simulink model "Supplementary_With_Disturbance"  (R2021a)
(part 42 of 51)

                                                                                                                                                                                                                                                                                                                                                                                                                                                                                                                                                                                                                                                                                                                                                                                                                                                                                                                                                                                                                                                                                                                                                                                                                                                                                                                                                                                                                                                                                                                                                                                                                                                                                                                                                                                                                                                                                                                                                                                                                                                                                                                                                                                                                                                                                                                                                                                                                                                                                                                                                                                                                                                                                                                                                                                                                                                                                                                                                                                                                                                                                                                                                                                                                                                                                                                                                                                                                                                                                                                                                                                                                                                                                                                                                                                                                                                                                                                                                                                                                                                                                                                                                                                                                                                                                                                                                                                                                                                                                                                                                                                                                                                                                                                                                                                                                                                                                                                                                                                                                                                                                                                                                                                                                                                                                                                                                                                                                                                                                                                                                                                                                                                                                                                                                                                                                                                                                                                                                                                                                                                                                                                                                                                                                                                                                                                                                                                                                                                                                                                                                                                                                                                                                                                                                                                                                                                                                                                                                                                                                                                                                                                                                                                                                                                                                                                                                                                                                                                                                                                                                                                                                                                                                                                                                                                                                                                                                                                                                                                                                                                                                                                                                                                                                                                                                                                                                                                                                                                                                                                                                                                                                                                                                                                                                                                                                                                                                                                                                                                                                                                                                                                                                                                                                                                                                                                                                                                                                                                                                                                                                                                                                                                                                                                                                                                                                                                                                                                                                                                                                                                                                                                                                                                                                                                                                                                                                                                                                                                                                                                                                                                                                                                                                                                                                                                                                                                                                                                                                                                                             0.5*I_yz_4*cos(theta3 - theta2 + theta4) + (I_xz_4*sin(theta3 - theta2 + theta4))/2 - 0.5*I_xz_5*cos(theta2 + theta3 + theta4 + theta5) + 0.5*I_yz_5*sin(theta2 + theta3 + theta4 + theta5) + I_zz_4*sin(theta2) + I_zz_5*sin(theta2) - 0.5*I_xz_5*cos(theta3 - theta2 + theta4 + theta5) + 0.5*I_yz_5*sin(theta3 - theta2 + theta4 + theta5) + 0.5*I_yz_4*cos(theta2 + theta3 + theta4) + (I_xz_4*sin(theta2 + theta3 + theta4))/2 + 0.25*a4^2*m4*sin(theta2) + a4^2*m5*sin(theta2) + 0.25*a5^2*m5*sin(theta2) + lc4_1^2*m4*sin(theta2) + lc4_2^2*m4*sin(theta2) + lc5_1^2*m5*sin(theta2) + lc5_2^2*m5*sin(theta2) - 0.25*a2*a4*m4*cos(theta3 - theta2 + theta4) - 0.5*a2*a4*m5*cos(theta3 - theta2 + theta4) + 0.25*a3*a5*m5*cos(theta4 - theta2 + theta5) - 0.5*a2*lc4_1*m4*cos(theta3 - theta2 + theta4) + (a3*lc5_1*m5*cos(theta4 - theta2 + theta5))/2 - 0.5*lc4_2*lc4_3*m4*cos(theta3 - theta2 + theta4) + 0.5*a2*lc4_2*m4*sin(theta3 - theta2 + theta4) - 0.25*a4*lc4_3*m4*sin(theta3 - theta2 + theta4) - 0.5*a3*lc5_2*m5*sin(theta4 - theta2 + theta5) - 0.5*a4*lc5_3*m5*sin(theta3 - theta2 + theta4) + 0.5*a2*lc5_2*m5*cos(theta2 + theta3 + theta4 + theta5) + 0.25*a5*lc5_3*m5*cos(theta2 + theta3 + theta4 + theta5) + 0.25*a2*a5*m5*sin(theta2 + theta3 + theta4 + theta5) - 0.5*lc4_1*lc4_3*m4*sin(theta3 - theta2 + theta4) + 0.5*lc5_1*lc5_3*m5*cos(theta2 + theta3 + theta4 + theta5) - (a4*a5*m5*cos(theta2 + theta5))/2 + 0.5*a2*lc5_1*m5*sin(theta2 + theta3 + theta4 + theta5) - 1.0*a1*lc4_2*m4*cos(theta3 + theta4) + 0.5*a3*lc4_2*m4*cos(theta2 + theta4) - 1.0*a4*lc5_1*m5*cos(theta2 + theta5) - 0.5*lc5_2*lc5_3*m5*sin(theta2 + theta3 + theta4 + theta5) - 0.5*a1*a4*m4*sin(theta3 + theta4) - 1.0*a1*a4*m5*sin(theta3 + theta4) + 0.25*a3*a4*m4*sin(theta2 + theta4) + (a3*a4*m5*sin(theta2 + theta4))/2 - 1.0*a1*lc4_1*m4*sin(theta3 + theta4) + (a3*lc4_1*m4*sin(theta2 + theta4))/2 + 1.0*a4*lc5_2*m5*sin(theta2 + theta5) + a4*lc4_1*m4*sin(theta2) + a5*lc5_1*m5*sin(theta2) - 0.5*a2*lc5_2*m5*cos(theta3 - theta2 + theta4 + theta5) + 0.25*a5*lc5_3*m5*cos(theta3 - theta2 + theta4 + theta5) - 0.25*a2*a5*m5*sin(theta3 - theta2 + theta4 + theta5) + 0.5*lc5_1*lc5_3*m5*cos(theta3 - theta2 + theta4 + theta5) + (a4*a5*m5*cos(theta2 - theta5))/2 - 0.5*a2*lc5_1*m5*sin(theta3 - theta2 + theta4 + theta5) - 0.5*a3*lc4_2*m4*cos(theta2 - theta4) + 1.0*a4*lc5_1*m5*cos(theta2 - theta5) - 0.5*lc5_2*lc5_3*m5*sin(theta3 - theta2 + theta4 + theta5) + 0.25*a3*a4*m4*sin(theta2 - theta4) + (a3*a4*m5*sin(theta2 - theta4))/2 + 0.25*a2*a4*m4*cos(theta2 + theta3 + theta4) + 0.5*a2*a4*m5*cos(theta2 + theta3 + theta4) + 0.5*a1*a5*m5*cos(theta3 + theta4 + theta5) - 0.25*a3*a5*m5*cos(theta2 + theta4 + theta5) + (a3*lc4_1*m4*sin(theta2 - theta4))/2 + 1.0*a4*lc5_2*m5*sin(theta2 - theta5) + 0.5*a2*lc4_1*m4*cos(theta2 + theta3 + theta4) + 1.0*a1*lc5_1*m5*cos(theta3 + theta4 + theta5) - (a3*lc5_1*m5*cos(theta2 + theta4 + theta5))/2 - 0.5*lc4_2*lc4_3*m4*cos(theta2 + theta3 + theta4) - 0.5*a2*lc4_2*m4*sin(theta2 + theta3 + theta4) - 0.25*a4*lc4_3*m4*sin(theta2 + theta3 + theta4) - 1.0*a1*lc5_2*m5*sin(theta3 + theta4 + theta5) + 0.5*a3*lc5_2*m5*sin(theta2 + theta4 + theta5) - 0.5*a4*lc5_3*m5*sin(theta2 + theta3 + theta4) - 0.5*lc4_1*lc4_3*m4*sin(theta2 + theta3 + theta4),                                                                                                                                                                                                                                                                                                                                                                                                                                                                                                                                                                                                                                                                                                                                                                                                                                                                                                                                                                                                                                                                                                                                                                                                                                                                                                                                                                                                                                                                                                                                                                                                                                                                                                                                                                                                                                                                                                                                                                                                                                                                                                                                                                                                                                                                                                                                                                                                                                                                                                                                                                                                                                                                                                                                                                                                                                                                                                                                                                                                                                                                                                                                                                                                                                                                                                                                                                                                                                                                                                                                                                                                                                                                                                                                                                                                                                                                                                                                                                                                                                                                                                                                                                                                                                                                                                                                                                                                                                                                                                                                                                                                                                                                                                                                                                                                                                                                                                                                                                                                                                                                                                                                                                                                                                                                                                                                                                                                                                                                                                                                                                                                                                                                                                                                                                                                                                                                                                                                                                                                                                                                                                                                                                                                                                                                                                                                                                                                                                                                                                                                                                                                                                                                                                                                                                                                                 I_yz_4*sin(theta3 + theta4) - 1.0*I_xz_4*cos(theta3 + theta4) - 1.0*I_yz_5*cos(theta3 + theta4 + theta5) - 1.0*I_xz_5*sin(theta3 + theta4 + theta5) + 0.5*a4*lc4_3*m4*cos(theta3 + theta4) + a4*lc5_3*m5*cos(theta3 + theta4) + lc4_1*lc4_3*m4*cos(theta3 + theta4) - 1.0*lc4_2*lc4_3*m4*sin(theta3 + theta4) + lc5_2*lc5_3*m5*cos(theta3 + theta4 + theta5) + 0.5*a5*lc5_3*m5*sin(theta3 + theta4 + theta5) + lc5_1*lc5_3*m5*sin(theta3 + theta4 + theta5),                                                                                                                                                                                                                                                                                                                                                                                                                                                                                                                                                                                                                                                                                                                                                                                                                                                                                                                                                                                                                                                                                                                                                                                                                                                                                                                                                                                                                                                                                                                                                                                                                                                                                                                                                                                                                                                                                                                                                                                                                                                                                                                                                                                                                                                                                                                                                                                                                                                                                                                                                                                                                                                                                                                                                                                                                                                                                                                                                                                                                                                                                                                                                                                                                                                                                                                                                                                                                                                                                                                                                                                                                                                                                                                                                                                                                                                                                                                                                                                                                                                                                                                  I_zz_4 + I_zz_5 + 0.25*a4^2*m4 + a4^2*m5 + 0.25*a5^2*m5 + lc4_1^2*m4 + lc4_2^2*m4 + lc5_1^2*m5 + lc5_2^2*m5 + a4*lc4_1*m4 + a5*lc5_1*m5 + a3*lc5_2*m5*cos(theta4 + theta5) + 0.5*a3*a5*m5*sin(theta4 + theta5) + a3*lc5_1*m5*sin(theta4 + theta5) + 0.5*a3*a4*m4*cos(theta4) + a3*a4*m5*cos(theta4) + a3*lc4_1*m4*cos(theta4) + 2.0*a4*lc5_2*m5*cos(theta5) + a4*a5*m5*sin(theta5) - 1.0*a3*lc4_2*m4*sin(theta4) + 2.0*a4*lc5_1*m5*sin(theta5),                                                                                                                                                                                                                                                                                                                                                                                                                                                                                                                                                                                                                                                                                                                                                                                                                                                                                                                                                                                                                                                                                                                                                                                                                                                                                                                                                                                                                                                                                                                                                                                                                                                                                                                                                                                                                                                                                                                                                                                                                                                                                                                                                                                                                                                                                                                                                                                                                                                                                                                                                                                                                                                                                                                                                                                                                                                                                                                                                                                                                                                                                                                         I_zz_4 + I_zz_5 + 0.25*a4^2*m4 + a4^2*m5 + 0.25*a5^2*m5 + lc4_1^2*m4 + lc4_2^2*m4 + lc5_1^2*m5 + lc5_2^2*m5 + a4*lc4_1*m4 + a5*lc5_1*m5 + 2.0*a4*lc5_2*m5*cos(theta5) + a4*a5*m5*sin(theta5) + 2.0*a4*lc5_1*m5*sin(theta5),                                                                                                                                                                                                                                                                                                                                                                                                                                                                                                                                                                                                                                                                                                                                                                                                                                                                                                                                                                                                                                                                                                                                                                                                                                                                                                                                                                                                                                                                                                                    0.25*m5*a5^2 + m5*a5*lc5_1 + 0.5*a4*m5*sin(theta5)*a5 + m5*lc5_1^2 + a4*m5*sin(theta5)*lc5_1 + m5*lc5_2^2 + a4*m5*cos(theta5)*lc5_2 + I_zz_5
                                                                                                                                                                                                                                                                                                                                                                                                                                                                                                                                                                                                                                                                                                                                                                                                                                                                                                                                                                                                                                                                                                                                                                                                                                                                                                                                                                                                                                                                                                                                                                                                                                                                                                                                                                                                                                                                                                                                                                                                                                                                                                                                                                                                                                                                                                                                                                                                                                                                                                                                                                                                                                                                                                                                                                                                                                                                                                                                                                                                                                                                                                                                                                                                                                                                                                                                                                                                                                                                                                                                                                                                                                                                                                                                                                                                                                                                                                                                                                                                                                                                                                                                                                                                                                                                                                                                                                                                                                                                                                                                                                                                                                                                                                                                                                                                                                                                                                                                                                                                                                                                                                                                                                                                                                                                                                                                                                                                                                                                                                                                                                                                                                                                                                                                                                                                                                                                                                                                                                                                                                                                                                                                                                                                                                                                                                                                                                                                                                                                                                                                                                                                                                                                                                                                                                                                                                                                                                                                                                                                                                                                                                                                                                                                                                                                                                                                                                                                                                                                                                                                                                                                                                                                                                                                                                                                                                                                                                                                                                                                                                                                                                                                                                                                                                                                                                                                                                                                                                                                                                                                                                                                                                                                                                                                                                                                                                                                                                                                                                                                                                                                                                                                                                                                                                                                                                                                                                                                                                                                                                                                                                                                                                                                                                                                                                                                                                                                                                                                                                                                                                                                                                                                                                                                                                                                                                                                                                                                                                                                                                                                                                                                                                                                                                                                                                                                                                                                                                                                                                                                                                                                                                                                                                                                                                                                                                                                                                                                                                                                                                                                                                                                                                                                                                                                                                                                                                                                                                                                                                                                                                                                                                                                                                                                                                                                                                                                                                                                                                                                                                                                                                                                                                                                                                0.5*I_yz_5*sin(theta2 + theta3 + theta4 + theta5) - 0.5*I_xz_5*cos(theta2 + theta3 + theta4 + theta5) + I_zz_5*sin(theta2) - 0.5*I_xz_5*cos(theta3 - theta2 + theta4 + theta5) + 0.5*I_yz_5*sin(theta3 - theta2 + theta4 + theta5) + 0.25*a5^2*m5*sin(theta2) + lc5_1^2*m5*sin(theta2) + lc5_2^2*m5*sin(theta2) + 0.25*a3*a5*m5*cos(theta4 - theta2 + theta5) + (a3*lc5_1*m5*cos(theta4 - theta2 + theta5))/2 - 0.5*a3*lc5_2*m5*sin(theta4 - theta2 + theta5) + 0.5*a2*lc5_2*m5*cos(theta2 + theta3 + theta4 + theta5) + 0.25*a5*lc5_3*m5*cos(theta2 + theta3 + theta4 + theta5) + 0.25*a2*a5*m5*sin(theta2 + theta3 + theta4 + theta5) + 0.5*lc5_1*lc5_3*m5*cos(theta2 + theta3 + theta4 + theta5) + 0.5*a2*lc5_1*m5*sin(theta2 + theta3 + theta4 + theta5) - 0.5*lc5_2*lc5_3*m5*sin(theta2 + theta3 + theta4 + theta5) + (a4*lc5_2*m5*sin(theta2 + theta5))/2 + a5*lc5_1*m5*sin(theta2) - 0.5*a2*lc5_2*m5*cos(theta3 - theta2 + theta4 + theta5) + 0.25*a5*lc5_3*m5*cos(theta3 - theta2 + theta4 + theta5) - 0.25*a2*a5*m5*sin(theta3 - theta2 + theta4 + theta5) + 0.5*lc5_1*lc5_3*m5*cos(theta3 - theta2 + theta4 + theta5) - 0.5*a2*lc5_1*m5*sin(theta3 - theta2 + theta4 + theta5) - 0.5*lc5_2*lc5_3*m5*sin(theta3 - theta2 + theta4 + theta5) + 0.5*a1*a5*m5*cos(theta3 + theta4 + theta5) - 0.25*a3*a5*m5*cos(theta2 + theta4 + theta5) + (a4*lc5_2*m5*sin(theta2 - theta5))/2 + a1*lc5_1*m5*cos(theta3 + theta4 + theta5) - (a3*lc5_1*m5*cos(theta2 + theta4 + theta5))/2 - 1.0*a1*lc5_2*m5*sin(theta3 + theta4 + theta5) + 0.5*a3*lc5_2*m5*sin(theta2 + theta4 + theta5) + 0.5*a4*a5*m5*sin(theta2)*sin(theta5) + a4*lc5_1*m5*sin(theta2)*sin(theta5),                                                                                                                                                                                                                                                                                                                                                                                                                                                                                                                                                                                                                                                                                                                                                                                                                                                                                                                                                                                                                                                                                                                                                                                                                                                                                                                                                                                                                                                                                                                                                                                                                                                                                                                                                                                                                                                                                                                                                                                                                                                                                                                                                                                                                                                                                                                                                                                                                                                                                                                                                                                                                                                                                                                                                                                                                                                                                                                                                                                                                                                                                                                                                                                                                                                                                                                                                                                                                                                                                                                                                                                                                                                                                                                                                                                                                                                                                                                                                                                                                                                                                                                                                                                                                                                                                                                                                                                                                                                                                                                                                                                                                                                                                                                                                                                                                                                                                                                                                                                                                                                                                                                                                                                                                                                                                                                                                                                                                                                                                                                                                                                                                                                                                                                                                                                                                                                                                                                                                                                                                                                                                                                                                                                                                                                                                                                                                                                                                                                                                                                                                                                                                                                                                                                                                                                                                                                                                                                                                                                                                                           lc5_2*lc5_3*m5*cos(theta3 + theta4 + theta5) - 1.0*I_xz_5*sin(theta3 + theta4 + theta5) - 1.0*I_yz_5*cos(theta3 + theta4 + theta5) + 0.5*a5*lc5_3*m5*sin(theta3 + theta4 + theta5) + lc5_1*lc5_3*m5*sin(theta3 + theta4 + theta5),                                                                                                                                                                                                                                                                                                                                                                                                                                                                                                                                                                                                                                                                                                                                                                                                                                                                                                                                                                                                                                                                                                                                                                                                                                                                                                                                                                                                                                                                                                                                                                                                                                                                                                                                                                                                                                                                                                                                                                                                                                                                                                                                                                                                                                                                                                                                                                                                                                                                                                                                                                                                                                                                                                                                                                                                                                                                                                                                                                                                                                                                                                                                                                                                                                                                                                                                                                                                                                                                                                                                                                                                                                                                                                                                                                                                                                                                                                                                                                                                                                                                                                                                                                                                                                                                                                          I_zz_5 + 0.25*a5^2*m5 + lc5_1^2*m5 + lc5_2^2*m5 + a5*lc5_1*m5 + a3*lc5_2*m5*cos(theta4 + theta5) + 0.5*a3*a5*m5*sin(theta4 + theta5) + a3*lc5_1*m5*sin(theta4 + theta5) + a4*lc5_2*m5*cos(theta5) + 0.5*a4*a5*m5*sin(theta5) + a4*lc5_1*m5*sin(theta5),                                                                                                                                                                                                                                                                                                                                                                                                                                                                                                                                                                                                                                                                                                                                                                                                                                                                                                                                                                                                                                                                                                                                                                                                                                                                                                                                                                                                                                                                                                                                                                                                                                                                                                                                                                                                                                                                                                                                                                                                                                                                                                                                                                                                                                                                                                                                                                                                                                                                                                                                                                                                                                                                                                                                                                                                                                                                                                                                                                                                                                                                                                                                                                                                       0.25*m5*a5^2 + m5*a5*lc5_1 + 0.5*a4*m5*sin(theta5)*a5 + m5*lc5_1^2 + a4*m5*sin(theta5)*lc5_1 + m5*lc5_2^2 + a4*m5*cos(theta5)*lc5_2 + I_zz_5,                                                                                                                                                                                                                                                                                                                                                                                                                                                                                                                                                                                                                                                                                                                                                                                                                                                                                                                                                                                                                                                                                                                                                                                                                                                                                                                                                                                                                                                                                                                                                                                                   0.25*m5*a5^2 + m5*a5*lc5_1 + m5*lc5_1^2 + m5*lc5_2^2 + I_zz_5]
 
%%%%%%%%%%%%%%%%%%%%%%%%%%%%%
% Coriolis and Centripetal Matrix
C11a = 0.5*I_yz_3*theta_dot_2*cos(2.0*theta2 - 1.0*theta3) - 0.25*I_yz_3*theta_dot_3*cos(2.0*theta2 - 1.0*theta3) - 0.5*I_xz_3*theta_dot_2*sin(2.0*theta2 - 1.0*theta3) + 0.25*I_xz_3*theta_dot_3*sin(2.0*theta2 - 1.0*theta3) - 0.25*I_xy_5*theta_dot_2*cos(2*theta2 + 2*theta3 + 2*theta4 + 2*theta5) - 0.25*I_xy_5*theta_dot_3*cos(2*theta2 + 2*theta3 + 2*theta4 + 2*theta5) - 0.25*I_xy_5*theta_dot_4*cos(2*theta2 + 2*theta3 + 2*theta4 + 2*theta5) - 0.25*I_xy_5*theta_dot_5*cos(2*theta2 + 2*theta3 + 2*theta4 + 2*theta5) - 0.125*I_xx_5*theta_dot_2*sin(2*theta2 + 2*theta3 + 2*theta4 + 2*theta5) - 0.125*I_xx_5*theta_dot_3*sin(2*theta2 + 2*theta3 + 2*theta4 + 2*theta5) - 0.125*I_xx_5*theta_dot_4*sin(2*theta2 + 2*theta3 + 2*theta4 + 2*theta5) - 0.125*I_xx_5*theta_dot_5*sin(2*theta2 + 2*theta3 + 2*theta4 + 2*theta5) + 0.125*I_yy_5*theta_dot_2*sin(2*theta2 + 2*theta3 + 2*theta4 + 2*theta5) + 0.125*I_yy_5*theta_dot_3*sin(2*theta2 + 2*theta3 + 2*theta4 + 2*theta5) + 0.125*I_yy_5*theta_dot_4*sin(2*theta2 + 2*theta3 + 2*theta4 + 2*theta5) + 0.125*I_yy_5*theta_dot_5*sin(2*theta2 + 2*theta3 + 2*theta4 + 2*theta5) - 0.5*I_xz_5*theta_dot_2*cos(theta3 - 2.0*theta2 + theta4 + theta5) - 0.5*I_xz_5*theta_dot_2*cos(2.0*theta2 + theta3 + theta4 + theta5) + 0.25*I_xz_5*theta_dot_3*cos(theta3 - 2.0*theta2 + theta4 + theta5) - 0.25*I_xz_5*theta_dot_3*cos(2.0*theta2 + theta3 + theta4 + theta5) + 0.25*I_xz_5*theta_dot_4*cos(theta3 - 2.0*theta2 + theta4 + theta5) - 0.25*I_xz_5*theta_dot_4*cos(2.0*theta2 + theta3 + theta4 + theta5) + 0.25*I_xz_5*theta_dot_5*cos(theta3 - 2.0*theta2 + theta4 + theta5) - 0.25*I_xz_5*theta_dot_5*cos(2.0*theta2 + theta3 + theta4 + theta5) + 0.25*I_xy_4*theta_dot_2*cos(2*theta2 + 2*theta3 + 2*theta4) + 0.25*I_xy_4*theta_dot_3*cos(2*theta2 + 2*theta3 + 2*theta4) + 0.25*I_xy_4*theta_dot_4*cos(2*theta2 + 2*theta3 + 2*theta4) - 0.5*I_xy_5*theta_dot_3*cos(2*theta3 + 2*theta4 + 2*theta5) - 0.5*I_xy_5*theta_dot_4*cos(2*theta3 + 2*theta4 + 2*theta5) - 0.5*I_xy_5*theta_dot_5*cos(2*theta3 + 2*theta4 + 2*theta5) + 0.5*I_yz_5*theta_dot_2*sin(theta3 - 2.0*theta2 + theta4 + theta5) + 0.5*I_yz_5*theta_dot_2*sin(2.0*theta2 + theta3 + theta4 + theta5) - 0.25*I_yz_5*theta_dot_3*sin(theta3 - 2.0*theta2 + theta4 + theta5) + 0.25*I_yz_5*theta_dot_3*sin(2.0*theta2 + theta3 + theta4 + theta5) - 0.25*I_yz_5*theta_dot_4*sin(theta3 - 2.0*theta2 + theta4 + theta5) + 0.25*I_yz_5*theta_dot_4*sin(2.0*theta2 + theta3 + theta4 + theta5) - 0.25*I_yz_5*theta_dot_5*sin(theta3 - 2.0*theta2 + theta4 + theta5) + 0.25*I_yz_5*theta_dot_5*sin(2.0*theta2 + theta3 + theta4 + theta5) + 0.5*I_yz_3*theta_dot_2*cos(2.0*theta2 + theta3) + 0.25*I_yz_3*theta_dot_3*cos(2.0*theta2 + theta3) + 0.125*I_xx_4*theta_dot_2*sin(2*theta2 + 2*theta3 + 2*theta4) + 0.125*I_xx_4*theta_dot_3*sin(2*theta2 + 2*theta3 + 2*theta4) + 0.125*I_xx_4*theta_dot_4*sin(2*theta2 + 2*theta3 + 2*theta4) - 0.25*I_xx_5*theta_dot_3*sin(2*theta3 + 2*theta4 + 2*theta5) - 0.25*I_xx_5*theta_dot_4*sin(2*theta3 + 2*theta4 + 2*theta5) - 0.25*I_xx_5*theta_dot_5*sin(2*theta3 + 2*theta4 + 2*theta5) - 0.125*I_yy_4*theta_dot_2*sin(2*theta2 + 2*theta3 + 2*theta4) - 0.125*I_yy_4*theta_dot_3*sin(2*theta2 + 2*theta3 + 2*theta4) - 0.125*I_yy_4*theta_dot_4*sin(2*theta2 + 2*theta3 + 2*theta4) + 0.25*I_yy_5*theta_dot_3*sin(2*theta3 + 2*theta4 + 2*theta5) + 0.25*I_yy_5*theta_dot_4*sin(2*theta3 + 2*theta4 + 2*theta5) + 0.25*I_yy_5*theta_dot_5*sin(2*theta3 + 2*theta4 + 2*theta5) + 0.5*I_xz_3*theta_dot_2*sin(2.0*theta2 + theta3) + 0.25*I_xz_3*theta_dot_3*sin(2.0*theta2 + theta3) + 0.25*I_xy_3*theta_dot_2*cos(2*theta2 + 2*theta3) + 0.25*I_xy_3*theta_dot_3*cos(2*theta2 + 2*theta3) + 0.5*I_xy_4*theta_dot_3*cos(2*theta3 + 2*theta4) + 0.5*I_xy_4*theta_dot_4*cos(2*theta3 + 2*theta4) - 1.0*I_xz_2*theta_dot_2*cos(2.0*theta2) + 0.5*I_xy_3*theta_dot_3*cos(2.0*theta3) + 0.125*I_xx_3*theta_dot_2*sin(2*theta2 + 2*theta3) + 0.125*I_xx_3*theta_dot_3*sin(2*theta2 + 2*theta3) + 0.25*I_xx_4*theta_dot_3*sin(2*theta3 + 2*theta4) + 0.25*I_xx_4*theta_dot_4*sin(2*theta3 + 2*theta4) - 0.125*I_yy_3*theta_dot_2*sin(2*theta2 + 2*theta3) - 0.125*I_yy_3*theta_dot_3*sin(2*theta2 + 2*theta3) - 0.25*I_yy_4*theta_dot_3*sin(2*theta3 + 2*theta4) - 0.25*I_yy_4*theta_dot_4*sin(2*theta3 + 2*theta4) - 0.5*I_xx_2*theta_dot_2*sin(2.0*theta2) - 0.25*I_xx_3*theta_dot_2*sin(2.0*theta2) - 0.25*I_xx_4*theta_dot_2*sin(2.0*theta2) + 0.25*I_xx_3*theta_dot_3*sin(2.0*theta3) - 0.25*I_xx_5*theta_dot_2*sin(2.0*theta2) - 0.25*I_yy_3*theta_dot_2*sin(2.0*theta2) - 0.25*I_yy_4*theta_dot_2*sin(2.0*theta2) - 0.25*I_yy_3*theta_dot_3*sin(2.0*theta3) - 0.25*I_yy_5*theta_dot_2*sin(2.0*theta2) + 0.5*I_zz_2*theta_dot_2*sin(2.0*theta2) + 0.5*I_zz_3*theta_dot_2*sin(2.0*theta2) + 0.5*I_zz_4*theta_dot_2*sin(2.0*theta2) + 0.5*I_zz_5*theta_dot_2*sin(2.0*theta2) - 0.25*I_xy_3*theta_dot_2*cos(2*theta2 - 2.0*theta3) + 0.25*I_xy_3*theta_dot_3*cos(2*theta2 - 2.0*theta3) + 0.125*I_xx_3*theta_dot_2*sin(2*theta2 - 2.0*theta3) - 0.125*I_xx_3*theta_dot_3*sin(2*theta2 - 2.0*theta3) - 0.125*I_yy_3*theta_dot_2*sin(2*theta2 - 2.0*theta3) + 0.125*I_yy_3*theta_dot_3*sin(2*theta2 - 2.0*theta3) - 0.25*I_xy_4*theta_dot_2*cos(2.0*theta3 - 2*theta2 + 2.0*theta4) + 0.25*I_xy_4*theta_dot_3*cos(2.0*theta3 - 2*theta2 + 2.0*theta4) + 0.25*I_xy_4*theta_dot_4*cos(2.0*theta3 - 2*theta2 + 2.0*theta4) + 0.5*I_yz_4*theta_dot_2*cos(theta3 - 2.0*theta2 + theta4) + 0.5*I_yz_4*theta_dot_2*cos(2.0*theta2 + theta3 + theta4) - 0.25*I_yz_4*theta_dot_3*cos(theta3 - 2.0*theta2 + theta4) + 0.25*I_yz_4*theta_dot_3*cos(2.0*theta2 + theta3 + theta4) - 0.25*I_yz_4*theta_dot_4*cos(theta3 - 2.0*theta2 + theta4) + 0.25*I_yz_4*theta_dot_4*cos(2.0*theta2 + theta3 + theta4) - 0.125*I_xx_4*theta_dot_2*sin(2.0*theta3 - 2*theta2 + 2.0*theta4) + 0.125*I_xx_4*theta_dot_3*sin(2.0*theta3 - 2*theta2 + 2.0*theta4) + 0.125*I_xx_4*theta_dot_4*sin(2.0*theta3 - 2*theta2 + 2.0*theta4) + 0.125*I_yy_4*theta_dot_2*sin(2.0*theta3 - 2*theta2 + 2.0*theta4) - 0.125*I_yy_4*theta_dot_3*sin(2.0*theta3 - 2*theta2 + 2.0*theta4) - 0.125*I_yy_4*theta_dot_4*sin(2.0*theta3 - 2*theta2 + 2.0*theta4) + 0.5*I_xz_4*theta_dot_2*sin(theta3 - 2.0*theta2 + theta4) + 0.5*I_xz_4*theta_dot_2*sin(2.0*theta2 + theta3 + theta4) - 0.25*I_xz_4*theta_dot_3*sin(theta3 - 2.0*theta2 + theta4) + 0.25*I_xz_4*theta_dot_3*sin(2.0*theta2 + theta3 + theta4) - 0.25*I_xz_4*theta_dot_4*sin(theta3 - 2.0*theta2 + theta4) + 0.25*I_xz_4*theta_dot_4*sin(2.0*theta2 + theta3 + theta4) + 0.25*I_xy_5*theta_dot_2*cos(2.0*theta3 - 2*theta2 + 2.0*theta4 + 2.0*theta5) - 0.25*I_xy_5*theta_dot_3*cos(2.0*theta3 - 2*theta2 + 2.0*theta4 + 2.0*theta5) - 0.25*I_xy_5*theta_dot_4*cos(2.0*theta3 - 2*theta2 + 2.0*theta4 + 2.0*theta5) - 0.25*I_xy_5*theta_dot_5*cos(2.0*theta3 - 2*theta2 + 2.0*theta4 + 2.0*theta5) + 0.125*I_xx_5*theta_dot_2*sin(2.0*theta3 - 2*theta2 + 2.0*theta4 + 2.0*theta5) - 0.125*I_xx_5*theta_dot_3*sin(2.0*theta3 - 2*theta2 + 2.0*theta4 + 2.0*theta5) - 0.125*I_xx_5*theta_dot_4*sin(2.0*theta3 - 2*theta2 + 2.0*theta4 + 2.0*theta5) - 0.125*I_xx_5*theta_dot_5*sin(2.0*theta3 - 2*theta2 + 2.0*theta4 + 2.0*theta5) - 0.125*I_yy_5*theta_dot_2*sin(2.0*theta3 - 2*theta2 + 2.0*theta4 + 2.0*theta5) + 0.125*I_yy_5*theta_dot_3*sin(2.0*theta3 - 2*theta2 + 2.0*theta4 + 2.0*theta5) + 0.125*I_yy_5*theta_dot_4*sin(2.0*theta3 - 2*theta2 + 2.0*theta4 + 2.0*theta5) + 0.125*I_yy_5*theta_dot_5*sin(2.0*theta3 - 2*theta2 + 2.0*theta4 + 2.0*theta5) + 0.03125*a5^2*m5*theta_dot_2*sin(2*theta2 + 2*theta3 + 2*theta4 + 2*theta5) + 0.03125*a5^2*m5*theta_dot_3*sin(2*theta2 + 2*theta3 + 2*theta4 + 2*theta5) + 0.03125*a5^2*m5*theta_dot_4*sin(2*theta2 + 2*theta3 + 2*theta4 + 2*theta5) + 0.03125*a5^2*m5*theta_dot_5*sin(2*theta2 + 2*theta3 + 2*theta4 + 2*theta5) + 0.125*lc5_1^2*m5*theta_dot_2*sin(2*theta2 + 2*theta3 + 2*theta4 + 2*theta5) + 0.125*lc5_1^2*m5*theta_dot_3*sin(2*theta2 + 2*theta3 + 2*theta4 + 2*theta5) - 0.125*lc5_2^2*m5*theta_dot_2*sin(2*theta2 + 2*theta3 + 2*theta4 + 2*theta5) + 0.125*lc5_1^2*m5*theta_dot_4*sin(2*theta2 + 2*theta3 + 2*theta4 + 2*theta5) - 0.125*lc5_2^2*m5*theta_dot_3*sin(2*theta2 + 2*theta3 + 2*theta4 + 2*theta5) + 0.125*lc5_1^2*m5*theta_dot_5*sin(2*theta2 + 2*theta3 + 2*theta4 + 2*theta5) - 0.125*lc5_2^2*m5*theta_dot_4*sin(2*theta2 + 2*theta3 + 2*theta4 + 2*theta5) - 0.125*lc5_2^2*m5*theta_dot_5*sin(2*theta2 + 2*theta3 + 2*theta4 + 2*theta5) - 0.03125*a4^2*m4*theta_dot_2*sin(2*theta2 + 2*theta3 + 2*theta4) - 0.03125*a4^2*m4*theta_dot_3*sin(2*theta2 + 2*theta3 + 2*theta4) - 0.125*a4^2*m5*theta_dot_2*sin(2*theta2 + 2*theta3 + 2*theta4) - 0.03125*a4^2*m4*theta_dot_4*sin(2*theta2 + 2*theta3 + 2*theta4) - 0.125*a4^2*m5*theta_dot_3*sin(2*theta2 + 2*theta3 + 2*theta4) - 0.125*a4^2*m5*theta_dot_4*sin(2*theta2 + 2*theta3 + 2*theta4) + 0.0625*a5^2*m5*theta_dot_3*sin(2*theta3 + 2*theta4 + 2*theta5) + 0.0625*a5^2*m5*theta_dot_4*sin(2*theta3 + 2*theta4 + 2*theta5) + 0.0625*a5^2*m5*theta_dot_5*sin(2*theta3 + 2*theta4 + 2*theta5) - 0.125*lc4_1^2*m4*theta_dot_2*sin(2*theta2 + 2*theta3 + 2*theta4) - 0.125*lc4_1^2*m4*theta_dot_3*sin(2*theta2 + 2*theta3 + 2*theta4) + 0.125*lc4_2^2*m4*theta_dot_2*sin(2*theta2 + 2*theta3 + 2*theta4) - 0.125*lc4_1^2*m4*theta_dot_4*sin(2*theta2 + 2*theta3 + 2*theta4) + 0.125*lc4_2^2*m4*theta_dot_3*sin(2*theta2 + 2*theta3 + 2*theta4) + 0.125*lc4_2^2*m4*theta_dot_4*sin(2*theta2 + 2*theta3 + 2*theta4) + 0.25*lc5_1^2*m5*theta_dot_3*sin(2*theta3 + 2*theta4 + 2*theta5) + 0.25*lc5_1^2*m5*theta_dot_4*sin(2*theta3 + 2*theta4 + 2*theta5) - 0.25*lc5_2^2*m5*theta_dot_3*sin(2*theta3 + 2*theta4 + 2*theta5) + 0.25*lc5_1^2*m5*theta_dot_5*sin(2*theta3 + 2*theta4 + 2*theta5) - 0.25*lc5_2^2*m5*theta_dot_4*sin(2*theta3 + 2*theta4 + 2*theta5) - 0.25*lc5_2^2*m5*theta_dot_5*sin(2*theta3 + 2*theta4 + 2*theta5) - 0.03125*a3^2*m3*theta_dot_2*sin(2*theta2 + 2*theta3) - 0.03125*a3^2*m3*theta_dot_3*sin(2*theta2 + 2*theta3) - 0.125*a3^2*m4*theta_dot_2*sin(2*theta2 + 2*theta3) - 0.125*a3^2*m4*theta_dot_3*sin(2*theta2 + 2*theta3) - 0.125*a3^2*m5*theta_dot_2*sin(2*theta2 + 2*theta3) - 0.125*a3^2*m5*theta_dot_3*sin(2*theta2 + 2*theta3) - 0.0625*a4^2*m4*theta_dot_3*sin(2*theta3 + 2*theta4) - 0.0625*a4^2*m4*theta_dot_4*sin(2*theta3 + 2*theta4) - 0.25*a4^2*m5*theta_dot_3*sin(2*theta3 + 2*theta4) - 0.25*a4^2*m5*theta_dot_4*sin(2*theta3 + 2*theta4) - 0.125*lc3_1^2*m3*theta_dot_2*sin(2*theta2 + 2*theta3) - 0.125*lc3_1^2*m3*theta_dot_3*sin(2*theta2 + 2*theta3) + 0.125*lc3_2^2*m3*theta_dot_2*sin(2*theta2 + 2*theta3) + 0.125*lc3_2^2*m3*theta_dot_3*sin(2*theta2 + 2*theta3) - 0.25*lc4_1^2*m4*theta_dot_3*sin(2*theta3 + 2*theta4) - 0.25*lc4_1^2*m4*theta_dot_4*sin(2*theta3 + 2*theta4) + 0.25*lc4_2^2*m4*theta_dot_3*sin(2*theta3 + 2*theta4) + 0.25*lc4_2^2*m4*theta_dot_4*sin(2*theta3 + 2*theta4) + 0.125*a2^2*m2*theta_dot_2*sin(2.0*theta2) + 0.5*a2^2*m3*theta_dot_2*sin(2.0*theta2) + 0.5*a2^2*m4*theta_dot_2*sin(2.0*theta2) + 0.0625*a3^2*m3*theta_dot_2*sin(2.0*theta2) + 0.5*a2^2*m5*theta_dot_2*sin(2.0*theta2) + 0.25*a3^2*m4*theta_dot_2*sin(2.0*theta2) - 0.0625*a3^2*m3*theta_dot_3*sin(2.0*theta3) + 0.25*a3^2*m5*theta_dot_2*sin(2.0*theta2) + 0.0625*a4^2*m4*theta_dot_2*sin(2.0*theta2) - 0.25*a3^2*m4*theta_dot_3*sin(2.0*theta3) + 0.25*a4^2*m5*theta_dot_2*sin(2.0*theta2) - 0.25*a3^2*m5*theta_dot_3*sin(2.0*theta3) + 0.0625*a5^2*m5*theta_dot_2*sin(2.0*theta2) + 0.5*lc2_1^2*m2*theta_dot_2*sin(2.0*theta2) - 0.5*lc2_3^2*m2*theta_dot_2*sin(2.0*theta2) + 0.25*lc3_1^2*m3*theta_dot_2*sin(2.0*theta2) + 0.25*lc3_2^2*m3*theta_dot_2*sin(2.0*theta2) - 0.25*lc3_1^2*m3*theta_dot_3*sin(2.0*theta3) - 0.5*lc3_3^2*m3*theta_dot_2*sin(2.0*theta2) + 0.25*lc3_2^2*m3*theta_dot_3*sin(2.0*theta3) + 0.25*lc4_1^2*m4*theta_dot_2*sin(2.0*theta2) + 0.25*lc4_2^2*m4*theta_dot_2*sin(2.0*theta2) - 0.5*lc4_3^2*m4*theta_dot_2*sin(2.0*theta2) + 0.25*lc5_1^2*m5*theta_dot_2*sin(2.0*theta2) + 0.25*lc5_2^2*m5*theta_dot_2*sin(2.0*theta2) - 0.5*lc5_3^2*m5*theta_dot_2*sin(2.0*theta2) - 0.03125*a3^2*m3*theta_dot_2*sin(2*theta2 - 2.0*theta3) + 0.03125*a3^2*m3*theta_dot_3*sin(2*theta2 - 2.0*theta3) - 0.125*a3^2*m4*theta_dot_2*sin(2*theta2 - 2.0*theta3) + 0.125*a3^2*m4*theta_dot_3*sin(2*theta2 - 2.0*theta3) - 0.125*a3^2*m5*theta_dot_2*sin(2*theta2 - 2.0*theta3) + 0.125*a3^2*m5*theta_dot_3*sin(2*theta2 - 2.0*theta3) - 0.125*lc3_1^2*m3*theta_dot_2*sin(2*theta2 - 2.0*theta3) + 0.125*lc3_1^2*m3*theta_dot_3*sin(2*theta2 - 2.0*theta3) + 0.125*lc3_2^2*m3*theta_dot_2*sin(2*theta2 - 2.0*theta3) - 0.125*lc3_2^2*m3*theta_dot_3*sin(2*theta2 - 2.0*theta3) + 0.03125*a4^2*m4*theta_dot_2*sin(2.0*theta3 - 2*theta2 + 2.0*theta4) - 0.03125*a4^2*m4*theta_dot_3*sin(2.0*theta3 - 2*theta2 + 2.0*theta4) + 0.125*a4^2*m5*theta_dot_2*sin(2.0*theta3 - 2*theta2 + 2.0*theta4) - 0.03125*a4^2*m4*theta_dot_4*sin(2.0*theta3 - 2*theta2 + 2.0*theta4) - 0.125*a4^2*m5*theta_dot_3*sin(2.0*theta3 - 2*theta2 + 2.0*theta4) - 0.125*a4^2*m5*theta_dot_4*sin(2.0*theta3 - 2*theta2 + 2.0*theta4) + 0.125*lc4_1^2*m4*theta_dot_2*sin(2.0*theta3 - 2*theta2 + 2.0*theta4) - 0.125*lc4_1^2*m4*theta_dot_3*sin(2.0*theta3 - 2*theta2 + 2.0*theta4) - 0.125*lc4_2^2*m4*theta_dot_2*sin(2.0*theta3 - 2*theta2 + 2.0*theta4) - 0.125*lc4_1^2*m4*theta_dot_4*sin(2.0*theta3 - 2*theta2 + 2.0*theta4) + 0.125*lc4_2^2*m4*theta_dot_3*sin(2.0*theta3 - 2*theta2 + 2.0*theta4) + 0.125*lc4_2^2*m4*theta_dot_4*sin(2.0*theta3 - 2*theta2 + 2.0*theta4) - 0.03125*a5^2*m5*theta_dot_2*sin(2.0*theta3 - 2*theta2 + 2.0*theta4 + 2.0*theta5) + 0.03125*a5^2*m5*theta_dot_3*sin(2.0*theta3 - 2*theta2 + 2.0*theta4 + 2.0*theta5) + 0.03125*a5^2*m5*theta_dot_4*sin(2.0*theta3 - 2*theta2 + 2.0*theta4 + 2.0*theta5) + 0.03125*a5^2*m5*theta_dot_5*sin(2.0*theta3 - 2*theta2 + 2.0*theta4 + 2.0*theta5) - 0.125*lc5_1^2*m5*theta_dot_2*sin(2.0*theta3 - 2*theta2 + 2.0*theta4 + 2.0*theta5) + 0.125*lc5_1^2*m5*theta_dot_3*sin(2.0*theta3 - 2*theta2 + 2.0*theta4 + 2.0*theta5) + 0.125*lc5_2^2*m5*theta_dot_2*sin(2.0*theta3 - 2*theta2 + 2.0*theta4 + 2.0*theta5) + 0.125*lc5_1^2*m5*theta_dot_4*sin(2.0*theta3 - 2*theta2 + 2.0*theta4 + 2.0*theta5) - 0.125*lc5_2^2*m5*theta_dot_3*sin(2.0*theta3 - 2*theta2 + 2.0*theta4 + 2.0*theta5) + 0.125*lc5_1^2*m5*theta_dot_5*sin(2.0*theta3 - 2*theta2 + 2.0*theta4 + 2.0*theta5) - 0.125*lc5_2^2*m5*theta_dot_4*sin(2.0*theta3 - 2*theta2 + 2.0*theta4 + 2.0*theta5) - 0.125*lc5_2^2*m5*theta_dot_5*sin(2.0*theta3 - 2*theta2 + 2.0*theta4 + 2.0*theta5) + 0.5*a1*lc5_1*m5*theta_dot_2*cos(theta3 - theta2 + theta4 + theta5) - 0.5*a1*lc5_1*m5*theta_dot_3*cos(theta3 - theta2 + theta4 + theta5) - 0.5*a1*lc5_1*m5*theta_dot_4*cos(theta3 - theta2 + theta4 + theta5) - 0.5*a1*lc5_1*m5*theta_dot_5*cos(theta3 - theta2 + theta4 + theta5) - 0.5*lc3_2*lc3_3*m3*theta_dot_2*cos(2.0*theta2 - 1.0*theta3) + 0.25*lc3_2*lc3_3*m3*theta_dot_3*cos(2.0*theta2 - 1.0*theta3) - 0.5*a2*lc3_2*m3*theta_dot_2*sin(2.0*theta2 - 1.0*theta3) + 0.25*a2*lc3_2*m3*theta_dot_3*sin(2.0*theta2 - 1.0*theta3) + 0.25*a3*lc3_3*m3*theta_dot_2*sin(2.0*theta2 - 1.0*theta3) - 0.125*a3*lc3_3*m3*theta_dot_3*sin(2.0*theta2 - 1.0*theta3) + 0.25*a3*lc4_1*m4*theta_dot_2*sin(2.0*theta2 - 1.0*theta4) + 0.5*a3*lc4_3*m4*theta_dot_2*sin(2.0*theta2 - 1.0*theta3) - 0.125*a3*lc4_1*m4*theta_dot_4*sin(2.0*theta2 - 1.0*theta4) - 0.25*a3*lc4_3*m4*theta_dot_3*sin(2.0*theta2 - 1.0*theta3) + 0.5*a3*lc5_3*m5*theta_dot_2*sin(2.0*theta2 - 1.0*theta3) - 0.25*a3*lc5_3*m5*theta_dot_3*sin(2.0*theta2 - 1.0*theta3) + 0.25*a4*lc5_2*m5*theta_dot_2*sin(2.0*theta2 - 1.0*theta5) - 0.125*a4*lc5_2*m5*theta_dot_5*sin(2.0*theta2 - 1.0*theta5) - 0.5*a1*lc5_2*m5*theta_dot_2*sin(theta3 - theta2 + theta4 + theta5) + 0.5*a1*lc5_2*m5*theta_dot_3*sin(theta3 - theta2 + theta4 + theta5) + 0.5*a1*lc5_2*m5*theta_dot_4*sin(theta3 - theta2 + theta4 + theta5) + 0.5*a1*lc5_2*m5*theta_dot_5*sin(theta3 - theta2 + theta4 + theta5) + 0.5*lc3_1*lc3_3*m3*theta_dot_2*sin(2.0*theta2 - 1.0*theta3) - 0.25*lc3_1*lc3_3*m3*theta_dot_3*sin(2.0*theta2 - 1.0*theta3) + 0.125*a5*lc5_2*m5*theta_dot_2*cos(2*theta2 + 2*theta3 + 2*theta4 + 2*theta5) + 0.125*a5*lc5_2*m5*theta_dot_3*cos(2*theta2 + 2*theta3 + 2*theta4 + 2*theta5) + 0.125*a5*lc5_2*m5*theta_dot_4*cos(2*theta2 + 2*theta3 + 2*theta4 + 2*theta5) + 0.125*a5*lc5_2*m5*theta_dot_5*cos(2*theta2 + 2*theta3 + 2*theta4 + 2*theta5) + 0.25*lc5_1*lc5_2*m5*theta_dot_2*cos(2*theta2 + 2*theta3 + 2*theta4 + 2*theta5) + 0.25*lc5_1*lc5_2*m5*theta_dot_3*cos(2*theta2 + 2*theta3 + 2*theta4 + 2*theta5) + 0.25*lc5_1*lc5_2*m5*theta_dot_4*cos(2*theta2 + 2*theta3 + 2*theta4 + 2*theta5) + 0.25*lc5_1*lc5_2*m5*theta_dot_5*cos(2*theta2 + 2*theta3 + 2*theta4 + 2*theta5) - 0.5*a1*lc4_2*m4*theta_dot_2*cos(theta2 + theta3 + theta4) - 0.5*a1*lc4_2*m4*theta_dot_3*cos(theta2 + theta3 + theta4) - 0.5*a1*lc4_2*m4*theta_dot_4*cos(theta2 + theta3 + theta4) - 0.5*a2*lc5_2*m5*theta_dot_3*cos(theta3 + theta4 + theta5) - 0.5*a2*lc5_2*m5*theta_dot_4*cos(theta3 + theta4 + theta5) - 0.5*a2*lc5_2*m5*theta_dot_5*cos(theta3 + theta4 + theta5) + 0.125*a5*lc5_1*m5*theta_dot_2*sin(2*theta2 + 2*theta3 + 2*theta4 + 2*theta5) + 0.125*a5*lc5_1*m5*theta_dot_3*sin(2*theta2 + 2*theta3 + 2*theta4 + 2*theta5) + 0.125*a5*lc5_1*m5*theta_dot_4*sin(2*theta2 + 2*theta3 + 2*theta4 + 2*theta5) + 0.125*a5*lc5_1*m5*theta_dot_5*sin(2*theta2 + 2*theta3 + 2*theta4 + 2*theta5) - 0.25*a1*a4*m4*theta_dot_2*sin(theta2 + theta3 + theta4) - 0.25*a1*a4*m4*theta_dot_3*sin(theta2 + theta3 + theta4) - 0.5*a1*a4*m5*theta_dot_2*sin(theta2 + theta3 + theta4) - 0.25*a1*a4*m4*theta_dot_4*sin(theta2 + theta3 + theta4) - 0.5*a1*a4*m5*theta_dot_3*sin(theta2 + theta3 + theta4) - 0.5*a1*a4*m5*theta_dot_4*sin(theta2 + theta3 + theta4) - 0.25*a2*a5*m5*theta_dot_3*sin(theta3 + theta4 + theta5) - 0.25*a2*a5*m5*theta_dot_4*sin(theta3 + theta4 + theta5) - 0.25*a2*a5*m5*theta_dot_5*sin(theta3 + theta4 + theta5) - 0.5*a1*lc4_1*m4*theta_dot_2*sin(theta2 + theta3 + theta4) - 0.5*a1*lc4_1*m4*theta_dot_3*sin(theta2 + theta3 + theta4) - 0.5*a1*lc4_1*m4*theta_dot_4*sin(theta2 + theta3 + theta4) - 0.5*a2*lc5_1*m5*theta_dot_3*sin(theta3 + theta4 + theta5) - 0.5*a2*lc5_1*m5*theta_dot_4*sin(theta3 + theta4 + theta5) - 0.5*a2*lc5_1*m5*theta_dot_5*sin(theta3 + theta4 + theta5) - 0.5*a2*lc5_2*m5*theta_dot_2*cos(theta3 - 2.0*theta2 + theta4 + theta5) + 0.5*a2*lc5_2*m5*theta_dot_2*cos(2.0*theta2 + theta3 + theta4 + theta5) + 0.25*a2*lc5_2*m5*theta_dot_3*cos(theta3 - 2.0*theta2 + theta4 + theta5) + 0.25*a2*lc5_2*m5*theta_dot_3*cos(2.0*theta2 + theta3 + theta4 + theta5) + 0.25*a2*lc5_2*m5*theta_dot_4*cos(theta3 - 2.0*theta2 + theta4 + theta5) + 0.25*a2*lc5_2*m5*theta_dot_4*cos(2.0*theta2 + theta3 + theta4 + theta5) + 0.25*a2*lc5_2*m5*theta_dot_5*cos(theta3 - 2.0*theta2 + theta4 + theta5) + 0.25*a2*lc5_2*m5*theta_dot_5*cos(2.0*theta2 + theta3 + theta4 + theta5) + 0.25*a5*lc5_3*m5*theta_dot_2*cos(theta3 - 2.0*theta2 + theta4 + theta5) + 0.25*a5*lc5_3*m5*theta_dot_2*cos(2.0*theta2 + theta3 + theta4 + theta5) - 0.125*a5*lc5_3*m5*theta_dot_3*cos(theta3 - 2.0*theta2 + theta4 + theta5) + 0.125*a5*lc5_3*m5*theta_dot_3*cos(2.0*theta2 + theta3 + theta4 + theta5) - 0.125*a5*lc5_3*m5*theta_dot_4*cos(theta3 - 2.0*theta2 + theta4 + theta5) + 0.125*a5*lc5_3*m5*theta_dot_4*cos(2.0*theta2 + theta3 + theta4 + theta5) - 0.125*a5*lc5_3*m5*theta_dot_5*cos(theta3 - 2.0*theta2 + theta4 + theta5) + 0.125*a5*lc5_3*m5*theta_dot_5*cos(2.0*theta2 + theta3 + theta4 + theta5) - 0.25*a2*a5*m5*theta_dot_2*sin(theta3 - 2.0*theta2 + theta4 + theta5) + 0.25*a2*a5*m5*theta_dot_2*sin(2.0*theta2 + theta3 + theta4 + theta5) + 0.125*a2*a5*m5*theta_dot_3*sin(theta3 - 2.0*theta2 + theta4 + theta5) + 0.125*a2*a5*m5*theta_dot_3*sin(2.0*theta2 + theta3 + theta4 + theta5) + 0.125*a2*a5*m5*theta_dot_4*sin(theta3 - 2.0*theta2 + theta4 + theta5) + 0.125*a2*a5*m5*theta_dot_4*sin(2.0*theta2 + theta3 + theta4 + theta5) + 0.125*a2*a5*m5*theta_dot_5*sin(theta3 - 2.0*theta2 + theta4 + theta5) + 0.125*a2*a5*m5*theta_dot_5*sin(2.0*theta2 + theta3 + theta4 + theta5) - 0.125*a4*lc4_2*m4*theta_dot_2*cos(2*theta2 + 2*theta3 + 2*theta4) - 0.125*a4*lc4_2*m4*theta_dot_3*cos(2*theta2 + 2*theta3 + 2*theta4) - 0.125*a4*lc4_2*m4*theta_dot_4*cos(2*theta2 + 2*theta3 + 2*theta4) + 0.25*a5*lc5_2*m5*theta_dot_3*cos(2*theta3 + 2*theta4 + 2*theta5) + 0.25*a5*lc5_2*m5*theta_dot_4*cos(2*theta3 + 2*theta4 + 2*theta5) + 0.25*a5*lc5_2*m5*theta_dot_5*cos(2*theta3 + 2*theta4 + 2*theta5) + 0.5*lc5_1*lc5_3*m5*theta_dot_2*cos(theta3 - 2.0*theta2 + theta4 + theta5) + 0.5*lc5_1*lc5_3*m5*theta_dot_2*cos(2.0*theta2 + theta3 + theta4 + theta5) - 0.25*lc5_1*lc5_3*m5*theta_dot_3*cos(theta3 - 2.0*theta2 + theta4 + theta5) + 0.25*lc5_1*lc5_3*m5*theta_dot_3*cos(2.0*theta2 + theta3 + theta4 + theta5) - 0.25*lc5_1*lc5_3*m5*theta_dot_4*cos(theta3 - 2.0*theta2 + theta4 + theta5) + 0.25*lc5_1*lc5_3*m5*theta_dot_4*cos(2.0*theta2 + theta3 + theta4 + theta5) - 0.25*lc5_1*lc5_3*m5*theta_dot_5*cos(theta3 - 2.0*theta2 + theta4 + theta5) + 0.25*lc5_1*lc5_3*m5*theta_dot_5*cos(2.0*theta2 + theta3 + theta4 + theta5) + 0.25*a2*a3*m3*theta_dot_2*cos(2.0*theta2 + theta3) + 0.125*a2*a3*m3*theta_dot_3*cos(2.0*theta2 + theta3) + 0.5*a2*a3*m4*theta_dot_2*cos(2.0*theta2 + theta3) + 0.25*a2*a3*m4*theta_dot_3*cos(2.0*theta2 + theta3) + 0.5*a2*a3*m5*theta_dot_2*cos(2.0*theta2 + theta3) + 0.25*a2*a3*m5*theta_dot_3*cos(2.0*theta2 + theta3) - 0.125*a4*a5*m5*theta_dot_2*cos(2.0*theta2 + theta5) - 0.0625*a4*a5*m5*theta_dot_5*cos(2.0*theta2 + theta5) - 0.5*a2*lc5_1*m5*theta_dot_2*sin(theta3 - 2.0*theta2 + theta4 + theta5) + 0.5*a2*lc5_1*m5*theta_dot_2*sin(2.0*theta2 + theta3 + theta4 + theta5) + 0.25*a2*lc5_1*m5*theta_dot_3*sin(theta3 - 2.0*theta2 + theta4 + theta5) + 0.25*a2*lc5_1*m5*theta_dot_3*sin(2.0*theta2 + theta3 + theta4 + theta5) + 0.25*a2*lc5_1*m5*theta_dot_4*sin(theta3 - 2.0*theta2 + theta4 + theta5) + 0.25*a2*lc5_1*m5*theta_dot_4*sin(2.0*theta2 + theta3 + theta4 + theta5) + 0.25*a2*lc5_1*m5*theta_dot_5*sin(theta3 - 2.0*theta2 + theta4 + theta5) + 0.25*a2*lc5_1*m5*theta_dot_5*sin(2.0*theta2 + theta3 + theta4 + theta5) - 0.25*lc4_1*lc4_2*m4*theta_dot_2*cos(2*theta2 + 2*theta3 + 2*theta4) - 0.25*lc4_1*lc4_2*m4*theta_dot_3*cos(2*theta2 + 2*theta3 + 2*theta4) - 0.25*lc4_1*lc4_2*m4*theta_dot_4*cos(2*theta2 + 2*theta3 + 2*theta4) + 0.5*lc5_1*lc5_2*m5*theta_dot_3*cos(2*theta3 + 2*theta4 + 2*theta5) + 0.5*lc5_1*lc5_2*m5*theta_dot_4*cos(2*theta3 + 2*theta4 + 2*theta5) + 0.5*lc5_1*lc5_2*m5*theta_dot_5*cos(2*theta3 + 2*theta4 + 2*theta5) - 0.5*a1*lc3_2*m3*theta_dot_2*cos(theta2 - 1.0*theta3) + 0.5*a1*lc3_2*m3*theta_dot_3*cos(theta2 - 1.0*theta3) + 0.5*a2*lc3_1*m3*theta_dot_2*cos(2.0*theta2 + theta3) + 0.25*a2*lc3_1*m3*theta_dot_3*cos(2.0*theta2 + theta3) + 0.25*a3*lc4_2*m4*theta_dot_2*cos(2.0*theta2 + theta4) - 0.5*a3*lc4_2*m4*theta_dot_3*cos(2.0*theta3 + theta4) + 0.125*a3*lc4_2*m4*theta_dot_4*cos(2.0*theta2 + theta4) - 0.25*a3*lc4_2*m4*theta_dot_4*cos(2.0*theta3 + theta4) - 0.25*a4*lc5_1*m5*theta_dot_2*cos(2.0*theta2 + theta5) - 0.125*a4*lc5_1*m5*theta_dot_5*cos(2.0*theta2 + theta5) - 0.125*a4*lc4_1*m4*theta_dot_2*sin(2*theta2 + 2*theta3 + 2*theta4) - 0.125*a4*lc4_1*m4*theta_dot_3*sin(2*theta2 + 2*theta3 + 2*theta4) - 0.125*a4*lc4_1*m4*theta_dot_4*sin(2*theta2 + 2*theta3 + 2*theta4) + 0.25*a5*lc5_1*m5*theta_dot_3*sin(2*theta3 + 2*theta4 + 2*theta5) + 0.25*a5*lc5_1*m5*theta_dot_4*sin(2*theta3 + 2*theta4 + 2*theta5) + 0.25*a5*lc5_1*m5*theta_dot_5*sin(2*theta3 + 2*theta4 + 2*theta5) - 0.5*lc5_2*lc5_3*m5*theta_dot_2*sin(theta3 - 2.0*theta2 + theta4 + theta5) - 0.5*lc5_2*lc5_3*m5*theta_dot_2*sin(2.0*theta2 + theta3 + theta4 + theta5) + 0.25*lc5_2*lc5_3*m5*theta_dot_3*sin(theta3 - 2.0*theta2 + theta4 + theta5) - 0.25*lc5_2*lc5_3*m5*theta_dot_3*sin(2.0*theta2 + theta3 + theta4 + theta5) + 0.25*lc5_2*lc5_3*m5*theta_dot_4*sin(theta3 - 2.0*theta2 + theta4 + theta5) - 0.25*lc5_2*lc5_3*m5*theta_dot_4*sin(2.0*theta2 + theta3 + theta4 + theta5) + 0.25*lc5_2*lc5_3*m5*theta_dot_5*sin(theta3 - 2.0*theta2 + theta4 + theta5) - 0.25*lc5_2*lc5_3*m5*theta_dot_5*sin(2.0*theta2 + theta3 + theta4 + theta5) + 0.25*a1*a3*m3*theta_dot_2*sin(theta2 - 1.0*theta3) - 0.25*a1*a3*m3*theta_dot_3*sin(theta2 - 1.0*theta3) + 0.5*a1*a3*m4*theta_dot_2*sin(theta2 - 1.0*theta3) - 0.5*a1*a3*m4*theta_dot_3*sin(theta2 - 1.0*theta3) + 0.5*a1*a3*m5*theta_dot_2*sin(theta2 - 1.0*theta3) - 0.5*a1*a3*m5*theta_dot_3*sin(theta2 - 1.0*theta3) + 0.125*a3*a4*m4*theta_dot_2*sin(2.0*theta2 + theta4) + 0.25*a3*a4*m5*theta_dot_2*sin(2.0*theta2 + theta4) - 0.25*a3*a4*m4*theta_dot_3*sin(2.0*theta3 + theta4) + 0.0625*a3*a4*m4*theta_dot_4*sin(2.0*theta2 + theta4) - 0.125*a3*a4*m4*theta_dot_4*sin(2.0*theta3 + theta4) - 0.5*a3*a4*m5*theta_dot_3*sin(2.0*theta3 + theta4) + 0.125*a3*a4*m5*theta_dot_4*sin(2.0*theta2 + theta4) - 0.25*a3*a4*m5*theta_dot_4*sin(2.0*theta3 + theta4) + 0.25*a4*a5*m5*theta_dot_3*cos(2.0*theta3 + 2.0*theta4 + theta5) + 0.25*a4*a5*m5*theta_dot_4*cos(2.0*theta3 + 2.0*theta4 + theta5) + 0.125*a4*a5*m5*theta_dot_5*cos(2.0*theta3 + 2.0*theta4 + theta5) - 0.5*lc3_2*lc3_3*m3*theta_dot_2*cos(2.0*theta2 + theta3) - 0.25*lc3_2*lc3_3*m3*theta_dot_3*cos(2.0*theta2 + theta3) + 0.5*a1*lc3_1*m3*theta_dot_2*sin(theta2 - 1.0*theta3) - 0.5*a1*lc3_1*m3*theta_dot_3*sin(theta2 - 1.0*theta3) - 0.5*a2*lc3_2*m3*theta_dot_2*sin(2.0*theta2 + theta3) - 0.25*a2*lc3_2*m3*theta_dot_3*sin(2.0*theta2 + theta3) - 0.25*a3*lc3_3*m3*theta_dot_2*sin(2.0*theta2 + theta3) - 0.125*a3*lc3_3*m3*theta_dot_3*sin(2.0*theta2 + theta3) + 0.25*a3*lc4_1*m4*theta_dot_2*sin(2.0*theta2 + theta4) - 0.5*a3*lc4_3*m4*theta_dot_2*sin(2.0*theta2 + theta3) - 0.5*a3*lc4_1*m4*theta_dot_3*sin(2.0*theta3 + theta4) + 0.125*a3*lc4_1*m4*theta_dot_4*sin(2.0*theta2 + theta4) - 0.25*a3*lc4_3*m4*theta_dot_3*sin(2.0*theta2 + theta3) - 0.25*a3*lc4_1*m4*theta_dot_4*sin(2.0*theta3 + theta4) - 0.5*a3*lc5_3*m5*theta_dot_2*sin(2.0*theta2 + theta3) - 0.25*a3*lc5_3*m5*theta_dot_3*sin(2.0*theta2 + theta3) + 0.25*a4*lc5_2*m5*theta_dot_2*sin(2.0*theta2 + theta5) + 0.125*a4*lc5_2*m5*theta_dot_5*sin(2.0*theta2 + theta5) + 0.25*a3*lc4_2*m4*theta_dot_2*cos(2.0*theta3 - 2.0*theta2 + theta4) - 0.25*a3*lc4_2*m4*theta_dot_2*cos(2.0*theta2 + 2.0*theta3 + theta4) - 0.25*a3*lc4_2*m4*theta_dot_3*cos(2.0*theta3 - 2.0*theta2 + theta4) - 0.25*a3*lc4_2*m4*theta_dot_3*cos(2.0*theta2 + 2.0*theta3 + theta4) - 0.125*a3*lc4_2*m4*theta_dot_4*cos(2.0*theta3 - 2.0*theta2 + theta4) - 0.125*a3*lc4_2*m4*theta_dot_4*cos(2.0*theta2 + 2.0*theta3 + theta4) + 0.5*a4*lc5_1*m5*theta_dot_3*cos(2.0*theta3 + 2.0*theta4 + theta5) 
C11b = 0.5*a4*lc5_1*m5*theta_dot_4*cos(2.0*theta3 + 2.0*theta4 + theta5) + 0.25*a4*lc5_1*m5*theta_dot_5*cos(2.0*theta3 + 2.0*theta4 + theta5) + 0.125*a3*a4*m4*theta_dot_2*sin(2.0*theta3 - 2.0*theta2 + theta4) - 0.125*a3*a4*m4*theta_dot_2*sin(2.0*theta2 + 2.0*theta3 + theta4) - 0.125*a3*a4*m4*theta_dot_3*sin(2.0*theta3 - 2.0*theta2 + theta4) - 0.125*a3*a4*m4*theta_dot_3*sin(2.0*theta2 + 2.0*theta3 + theta4) + 0.25*a3*a4*m5*theta_dot_2*sin(2.0*theta3 - 2.0*theta2 + theta4) - 0.25*a3*a4*m5*theta_dot_2*sin(2.0*theta2 + 2.0*theta3 + theta4) - 0.0625*a3*a4*m4*theta_dot_4*sin(2.0*theta3 - 2.0*theta2 + theta4) - 0.0625*a3*a4*m4*theta_dot_4*sin(2.0*theta2 + 2.0*theta3 + theta4) - 0.25*a3*a4*m5*theta_dot_3*sin(2.0*theta3 - 2.0*theta2 + theta4) - 0.25*a3*a4*m5*theta_dot_3*sin(2.0*theta2 + 2.0*theta3 + theta4) - 0.125*a3*a4*m5*theta_dot_4*sin(2.0*theta3 - 2.0*theta2 + theta4) - 0.125*a3*a4*m5*theta_dot_4*sin(2.0*theta2 + 2.0*theta3 + theta4) - 0.5*lc3_1*lc3_3*m3*theta_dot_2*sin(2.0*theta2 + theta3) - 0.25*lc3_1*lc3_3*m3*theta_dot_3*sin(2.0*theta2 + theta3) - 0.125*a4*a5*m5*theta_dot_2*cos(2.0*theta3 - 2.0*theta2 + 2.0*theta4 + theta5) + 0.125*a4*a5*m5*theta_dot_2*cos(2.0*theta2 + 2.0*theta3 + 2.0*theta4 + theta5) + 0.125*a4*a5*m5*theta_dot_3*cos(2.0*theta3 - 2.0*theta2 + 2.0*theta4 + theta5) + 0.125*a4*a5*m5*theta_dot_3*cos(2.0*theta2 + 2.0*theta3 + 2.0*theta4 + theta5) + 0.125*a4*a5*m5*theta_dot_4*cos(2.0*theta3 - 2.0*theta2 + 2.0*theta4 + theta5) + 0.125*a4*a5*m5*theta_dot_4*cos(2.0*theta2 + 2.0*theta3 + 2.0*theta4 + theta5) + 0.0625*a4*a5*m5*theta_dot_5*cos(2.0*theta3 - 2.0*theta2 + 2.0*theta4 + theta5) + 0.0625*a4*a5*m5*theta_dot_5*cos(2.0*theta2 + 2.0*theta3 + 2.0*theta4 + theta5) - 0.125*a3*lc3_2*m3*theta_dot_2*cos(2*theta2 + 2*theta3) - 0.125*a3*lc3_2*m3*theta_dot_3*cos(2*theta2 + 2*theta3) - 0.25*a4*lc4_2*m4*theta_dot_3*cos(2*theta3 + 2*theta4) - 0.25*a4*lc4_2*m4*theta_dot_4*cos(2*theta3 + 2*theta4) + 0.25*a3*lc4_1*m4*theta_dot_2*sin(2.0*theta3 - 2.0*theta2 + theta4) - 0.25*a3*lc4_1*m4*theta_dot_2*sin(2.0*theta2 + 2.0*theta3 + theta4) - 0.25*a3*lc4_1*m4*theta_dot_3*sin(2.0*theta3 - 2.0*theta2 + theta4) - 0.25*a3*lc4_1*m4*theta_dot_3*sin(2.0*theta2 + 2.0*theta3 + theta4) - 0.125*a3*lc4_1*m4*theta_dot_4*sin(2.0*theta3 - 2.0*theta2 + theta4) - 0.125*a3*lc4_1*m4*theta_dot_4*sin(2.0*theta2 + 2.0*theta3 + theta4) - 0.5*a4*lc5_2*m5*theta_dot_3*sin(2.0*theta3 + 2.0*theta4 + theta5) - 0.5*a4*lc5_2*m5*theta_dot_4*sin(2.0*theta3 + 2.0*theta4 + theta5) - 0.25*a4*lc5_2*m5*theta_dot_5*sin(2.0*theta3 + 2.0*theta4 + theta5) - 0.25*a4*lc5_1*m5*theta_dot_2*cos(2.0*theta3 - 2.0*theta2 + 2.0*theta4 + theta5) + 0.25*a4*lc5_1*m5*theta_dot_2*cos(2.0*theta2 + 2.0*theta3 + 2.0*theta4 + theta5) + 0.25*a4*lc5_1*m5*theta_dot_3*cos(2.0*theta3 - 2.0*theta2 + 2.0*theta4 + theta5) + 0.25*a4*lc5_1*m5*theta_dot_3*cos(2.0*theta2 + 2.0*theta3 + 2.0*theta4 + theta5) + 0.25*a4*lc5_1*m5*theta_dot_4*cos(2.0*theta3 - 2.0*theta2 + 2.0*theta4 + theta5) + 0.25*a4*lc5_1*m5*theta_dot_4*cos(2.0*theta2 + 2.0*theta3 + 2.0*theta4 + theta5) + 0.125*a4*lc5_1*m5*theta_dot_5*cos(2.0*theta3 - 2.0*theta2 + 2.0*theta4 + theta5) + 0.125*a4*lc5_1*m5*theta_dot_5*cos(2.0*theta2 + 2.0*theta3 + 2.0*theta4 + theta5) - 0.25*lc3_1*lc3_2*m3*theta_dot_2*cos(2*theta2 + 2*theta3) - 0.25*lc3_1*lc3_2*m3*theta_dot_3*cos(2*theta2 + 2*theta3) - 0.5*lc4_1*lc4_2*m4*theta_dot_3*cos(2*theta3 + 2*theta4) - 0.5*lc4_1*lc4_2*m4*theta_dot_4*cos(2*theta3 + 2*theta4) + 0.5*a2*lc2_3*m2*theta_dot_2*cos(2.0*theta2) + a2*lc3_3*m3*theta_dot_2*cos(2.0*theta2) - 0.25*a3*lc3_2*m3*theta_dot_3*cos(2.0*theta3) + a2*lc4_3*m4*theta_dot_2*cos(2.0*theta2) + a2*lc5_3*m5*theta_dot_2*cos(2.0*theta2) - 0.125*a3*lc3_1*m3*theta_dot_2*sin(2*theta2 + 2*theta3) - 0.125*a3*lc3_1*m3*theta_dot_3*sin(2*theta2 + 2*theta3) - 0.25*a4*lc4_1*m4*theta_dot_3*sin(2*theta3 + 2*theta4) - 0.25*a4*lc4_1*m4*theta_dot_4*sin(2*theta3 + 2*theta4) - 0.5*a1*lc4_2*m4*theta_dot_2*cos(theta3 - theta2 + theta4) + 0.5*a1*lc4_2*m4*theta_dot_3*cos(theta3 - theta2 + theta4) + 0.5*a1*lc4_2*m4*theta_dot_4*cos(theta3 - theta2 + theta4) + lc2_1*lc2_3*m2*theta_dot_2*cos(2.0*theta2) - 0.5*lc3_1*lc3_2*m3*theta_dot_3*cos(2.0*theta3) + 0.25*a4*lc5_2*m5*theta_dot_2*sin(2.0*theta3 - 2.0*theta2 + 2.0*theta4 + theta5) - 0.25*a4*lc5_2*m5*theta_dot_2*sin(2.0*theta2 + 2.0*theta3 + 2.0*theta4 + theta5) - 0.25*a4*lc5_2*m5*theta_dot_3*sin(2.0*theta3 - 2.0*theta2 + 2.0*theta4 + theta5) - 0.25*a4*lc5_2*m5*theta_dot_3*sin(2.0*theta2 + 2.0*theta3 + 2.0*theta4 + theta5) - 0.25*a4*lc5_2*m5*theta_dot_4*sin(2.0*theta3 - 2.0*theta2 + 2.0*theta4 + theta5) - 0.25*a4*lc5_2*m5*theta_dot_4*sin(2.0*theta2 + 2.0*theta3 + 2.0*theta4 + theta5) - 0.125*a4*lc5_2*m5*theta_dot_5*sin(2.0*theta3 - 2.0*theta2 + 2.0*theta4 + theta5) - 0.125*a4*lc5_2*m5*theta_dot_5*sin(2.0*theta2 + 2.0*theta3 + 2.0*theta4 + theta5) - 0.25*a1*a4*m4*theta_dot_2*sin(theta3 - theta2 + theta4) + 0.25*a1*a4*m4*theta_dot_3*sin(theta3 - theta2 + theta4) - 0.5*a1*a4*m5*theta_dot_2*sin(theta3 - theta2 + theta4) + 0.25*a1*a4*m4*theta_dot_4*sin(theta3 - theta2 + theta4) + 0.5*a1*a4*m5*theta_dot_3*sin(theta3 - theta2 + theta4) + 0.5*a1*a4*m5*theta_dot_4*sin(theta3 - theta2 + theta4) + 0.5*a2*lc2_1*m2*theta_dot_2*sin(2.0*theta2) + 0.25*a3*lc3_1*m3*theta_dot_2*sin(2.0*theta2) - 0.25*a3*lc3_1*m3*theta_dot_3*sin(2.0*theta3) + 0.25*a4*lc4_1*m4*theta_dot_2*sin(2.0*theta2) + 0.25*a5*lc5_1*m5*theta_dot_2*sin(2.0*theta2) + 0.25*a1*a5*m5*theta_dot_2*cos(theta2 + theta3 + theta4 + theta5) + 0.25*a1*a5*m5*theta_dot_3*cos(theta2 + theta3 + theta4 + theta5) + 0.25*a1*a5*m5*theta_dot_4*cos(theta2 + theta3 + theta4 + theta5) + 0.25*a1*a5*m5*theta_dot_5*cos(theta2 + theta3 + theta4 + theta5) - 0.5*a1*lc4_1*m4*theta_dot_2*sin(theta3 - theta2 + theta4) + 0.5*a1*lc4_1*m4*theta_dot_3*sin(theta3 - theta2 + theta4) + 0.5*a1*lc4_1*m4*theta_dot_4*sin(theta3 - theta2 + theta4) + 0.5*a1*lc5_1*m5*theta_dot_2*cos(theta2 + theta3 + theta4 + theta5) + 0.5*a1*lc5_1*m5*theta_dot_3*cos(theta2 + theta3 + theta4 + theta5) + 0.5*a1*lc5_1*m5*theta_dot_4*cos(theta2 + theta3 + theta4 + theta5) + 0.5*a1*lc5_1*m5*theta_dot_5*cos(theta2 + theta3 + theta4 + theta5) - 0.25*a2*a4*m4*theta_dot_3*cos(theta3 + theta4) - 0.25*a2*a4*m4*theta_dot_4*cos(theta3 + theta4) - 0.5*a2*a4*m5*theta_dot_3*cos(theta3 + theta4) - 0.5*a2*a4*m5*theta_dot_4*cos(theta3 + theta4) + 0.375*a3*a5*m5*theta_dot_4*cos(theta4 + theta5) + 0.375*a3*a5*m5*theta_dot_5*cos(theta4 + theta5) - 0.5*a1*lc5_2*m5*theta_dot_2*sin(theta2 + theta3 + theta4 + theta5) - 0.5*a1*lc5_2*m5*theta_dot_3*sin(theta2 + theta3 + theta4 + theta5) - 0.5*a1*lc5_2*m5*theta_dot_4*sin(theta2 + theta3 + theta4 + theta5) - 0.5*a1*lc5_2*m5*theta_dot_5*sin(theta2 + theta3 + theta4 + theta5) + 0.125*a3*lc3_2*m3*theta_dot_2*cos(2*theta2 - 2.0*theta3) - 0.125*a3*lc3_2*m3*theta_dot_3*cos(2*theta2 - 2.0*theta3) - 0.5*a1*lc3_2*m3*theta_dot_2*cos(theta2 + theta3) - 0.5*a1*lc3_2*m3*theta_dot_3*cos(theta2 + theta3) - 0.5*a2*lc4_1*m4*theta_dot_3*cos(theta3 + theta4) - 0.5*a2*lc4_1*m4*theta_dot_4*cos(theta3 + theta4) + 0.75*a3*lc5_1*m5*theta_dot_4*cos(theta4 + theta5) + 0.75*a3*lc5_1*m5*theta_dot_5*cos(theta4 + theta5) - 0.25*a1*a3*m3*theta_dot_2*sin(theta2 + theta3) - 0.25*a1*a3*m3*theta_dot_3*sin(theta2 + theta3) - 0.5*a1*a3*m4*theta_dot_2*sin(theta2 + theta3) - 0.5*a1*a3*m4*theta_dot_3*sin(theta2 + theta3) - 0.5*a1*a3*m5*theta_dot_2*sin(theta2 + theta3) - 0.5*a1*a3*m5*theta_dot_3*sin(theta2 + theta3) - 0.25*a2*a4*m4*theta_dot_2*cos(theta3 - 2.0*theta2 + theta4) + 0.25*a2*a4*m4*theta_dot_2*cos(2.0*theta2 + theta3 + theta4) + 0.125*a2*a4*m4*theta_dot_3*cos(theta3 - 2.0*theta2 + theta4) + 0.125*a2*a4*m4*theta_dot_3*cos(2.0*theta2 + theta3 + theta4) - 0.5*a2*a4*m5*theta_dot_2*cos(theta3 - 2.0*theta2 + theta4) + 0.5*a2*a4*m5*theta_dot_2*cos(2.0*theta2 + theta3 + theta4) + 0.125*a2*a4*m4*theta_dot_4*cos(theta3 - 2.0*theta2 + theta4) + 0.125*a2*a4*m4*theta_dot_4*cos(2.0*theta2 + theta3 + theta4) + 0.25*a2*a4*m5*theta_dot_3*cos(theta3 - 2.0*theta2 + theta4) + 0.25*a2*a4*m5*theta_dot_3*cos(2.0*theta2 + theta3 + theta4) + 0.25*a2*a4*m5*theta_dot_4*cos(theta3 - 2.0*theta2 + theta4) + 0.25*a2*a4*m5*theta_dot_4*cos(2.0*theta2 + theta3 + theta4) + 0.125*a3*a5*m5*theta_dot_2*cos(theta4 - 2.0*theta2 + theta5) - 0.125*a3*a5*m5*theta_dot_2*cos(2.0*theta2 + theta4 + theta5) + 0.25*a3*a5*m5*theta_dot_3*cos(2.0*theta3 + theta4 + theta5) - 0.0625*a3*a5*m5*theta_dot_4*cos(theta4 - 2.0*theta2 + theta5) - 0.0625*a3*a5*m5*theta_dot_4*cos(2.0*theta2 + theta4 + theta5) + 0.125*a3*a5*m5*theta_dot_4*cos(2.0*theta3 + theta4 + theta5) - 0.0625*a3*a5*m5*theta_dot_5*cos(theta4 - 2.0*theta2 + theta5) - 0.0625*a3*a5*m5*theta_dot_5*cos(2.0*theta2 + theta4 + theta5) + 0.125*a3*a5*m5*theta_dot_5*cos(2.0*theta3 + theta4 + theta5) + 0.25*lc3_1*lc3_2*m3*theta_dot_2*cos(2*theta2 - 2.0*theta3) - 0.25*lc3_1*lc3_2*m3*theta_dot_3*cos(2*theta2 - 2.0*theta3) - 0.125*a3*lc3_1*m3*theta_dot_2*sin(2*theta2 - 2.0*theta3) + 0.125*a3*lc3_1*m3*theta_dot_3*sin(2*theta2 - 2.0*theta3) - 0.5*a1*lc3_1*m3*theta_dot_2*sin(theta2 + theta3) - 0.5*a1*lc3_1*m3*theta_dot_3*sin(theta2 + theta3) + 0.5*a2*lc4_2*m4*theta_dot_3*sin(theta3 + theta4) + 0.5*a2*lc4_2*m4*theta_dot_4*sin(theta3 + theta4) - 0.75*a3*lc5_2*m5*theta_dot_4*sin(theta4 + theta5) - 0.75*a3*lc5_2*m5*theta_dot_5*sin(theta4 + theta5) + 0.125*a4*lc4_2*m4*theta_dot_2*cos(2.0*theta3 - 2*theta2 + 2.0*theta4) - 0.125*a4*lc4_2*m4*theta_dot_3*cos(2.0*theta3 - 2*theta2 + 2.0*theta4) - 0.125*a4*lc4_2*m4*theta_dot_4*cos(2.0*theta3 - 2*theta2 + 2.0*theta4) - 0.5*a2*lc4_1*m4*theta_dot_2*cos(theta3 - 2.0*theta2 + theta4) + 0.5*a2*lc4_1*m4*theta_dot_2*cos(2.0*theta2 + theta3 + theta4) + 0.25*a2*lc4_1*m4*theta_dot_3*cos(theta3 - 2.0*theta2 + theta4) + 0.25*a2*lc4_1*m4*theta_dot_3*cos(2.0*theta2 + theta3 + theta4) + 0.25*a2*lc4_1*m4*theta_dot_4*cos(theta3 - 2.0*theta2 + theta4) + 0.25*a2*lc4_1*m4*theta_dot_4*cos(2.0*theta2 + theta3 + theta4) + 0.25*a3*lc5_1*m5*theta_dot_2*cos(theta4 - 2.0*theta2 + theta5) - 0.25*a3*lc5_1*m5*theta_dot_2*cos(2.0*theta2 + theta4 + theta5) + 0.5*a3*lc5_1*m5*theta_dot_3*cos(2.0*theta3 + theta4 + theta5) - 0.125*a3*lc5_1*m5*theta_dot_4*cos(theta4 - 2.0*theta2 + theta5) - 0.125*a3*lc5_1*m5*theta_dot_4*cos(2.0*theta2 + theta4 + theta5) + 0.25*a3*lc5_1*m5*theta_dot_4*cos(2.0*theta3 + theta4 + theta5) - 0.125*a3*lc5_1*m5*theta_dot_5*cos(theta4 - 2.0*theta2 + theta5) - 0.125*a3*lc5_1*m5*theta_dot_5*cos(2.0*theta2 + theta4 + theta5) + 0.25*a3*lc5_1*m5*theta_dot_5*cos(2.0*theta3 + theta4 + theta5) - 0.125*a3*a5*m5*theta_dot_2*cos(2.0*theta3 - 2.0*theta2 + theta4 + theta5) + 0.125*a3*a5*m5*theta_dot_2*cos(2.0*theta2 + 2.0*theta3 + theta4 + theta5) + 0.125*a3*a5*m5*theta_dot_3*cos(2.0*theta3 - 2.0*theta2 + theta4 + theta5) + 0.125*a3*a5*m5*theta_dot_3*cos(2.0*theta2 + 2.0*theta3 + theta4 + theta5) + 0.0625*a3*a5*m5*theta_dot_4*cos(2.0*theta3 - 2.0*theta2 + theta4 + theta5) + 0.0625*a3*a5*m5*theta_dot_4*cos(2.0*theta2 + 2.0*theta3 + theta4 + theta5) + 0.0625*a3*a5*m5*theta_dot_5*cos(2.0*theta3 - 2.0*theta2 + theta4 + theta5) + 0.0625*a3*a5*m5*theta_dot_5*cos(2.0*theta2 + 2.0*theta3 + theta4 + theta5) + 0.25*lc4_1*lc4_2*m4*theta_dot_2*cos(2.0*theta3 - 2*theta2 + 2.0*theta4) - 0.25*lc4_1*lc4_2*m4*theta_dot_3*cos(2.0*theta3 - 2*theta2 + 2.0*theta4) - 0.25*lc4_1*lc4_2*m4*theta_dot_4*cos(2.0*theta3 - 2*theta2 + 2.0*theta4) - 0.5*lc4_2*lc4_3*m4*theta_dot_2*cos(theta3 - 2.0*theta2 + theta4) - 0.5*lc4_2*lc4_3*m4*theta_dot_2*cos(2.0*theta2 + theta3 + theta4) + 0.25*lc4_2*lc4_3*m4*theta_dot_3*cos(theta3 - 2.0*theta2 + theta4) - 0.25*lc4_2*lc4_3*m4*theta_dot_3*cos(2.0*theta2 + theta3 + theta4) + 0.25*lc4_2*lc4_3*m4*theta_dot_4*cos(theta3 - 2.0*theta2 + theta4) - 0.25*lc4_2*lc4_3*m4*theta_dot_4*cos(2.0*theta2 + theta3 + theta4) + 0.5*a1*a2*m2*theta_dot_2*cos(theta2) + a1*a2*m3*theta_dot_2*cos(theta2) + a1*a2*m4*theta_dot_2*cos(theta2) + a1*a2*m5*theta_dot_2*cos(theta2) - 0.25*a2*a3*m3*theta_dot_3*cos(theta3) - 0.5*a2*a3*m4*theta_dot_3*cos(theta3) - 0.5*a2*a3*m5*theta_dot_3*cos(theta3) + 0.375*a4*a5*m5*theta_dot_5*cos(theta5) + 0.125*a4*lc4_1*m4*theta_dot_2*sin(2.0*theta3 - 2*theta2 + 2.0*theta4) - 0.125*a4*lc4_1*m4*theta_dot_3*sin(2.0*theta3 - 2*theta2 + 2.0*theta4) - 0.125*a4*lc4_1*m4*theta_dot_4*sin(2.0*theta3 - 2*theta2 + 2.0*theta4) + 0.5*a2*lc4_2*m4*theta_dot_2*sin(theta3 - 2.0*theta2 + theta4) - 0.5*a2*lc4_2*m4*theta_dot_2*sin(2.0*theta2 + theta3 + theta4) - 0.25*a2*lc4_2*m4*theta_dot_3*sin(theta3 - 2.0*theta2 + theta4) - 0.25*a2*lc4_2*m4*theta_dot_3*sin(2.0*theta2 + theta3 + theta4) - 0.25*a2*lc4_2*m4*theta_dot_4*sin(theta3 - 2.0*theta2 + theta4) - 0.25*a2*lc4_2*m4*theta_dot_4*sin(2.0*theta2 + theta3 + theta4) - 0.25*a4*lc4_3*m4*theta_dot_2*sin(theta3 - 2.0*theta2 + theta4) - 0.25*a4*lc4_3*m4*theta_dot_2*sin(2.0*theta2 + theta3 + theta4) + 0.125*a4*lc4_3*m4*theta_dot_3*sin(theta3 - 2.0*theta2 + theta4) - 0.125*a4*lc4_3*m4*theta_dot_3*sin(2.0*theta2 + theta3 + theta4) + 0.125*a4*lc4_3*m4*theta_dot_4*sin(theta3 - 2.0*theta2 + theta4) - 0.125*a4*lc4_3*m4*theta_dot_4*sin(2.0*theta2 + theta3 + theta4) - 0.25*a3*lc5_2*m5*theta_dot_2*sin(theta4 - 2.0*theta2 + theta5) + 0.25*a3*lc5_2*m5*theta_dot_2*sin(2.0*theta2 + theta4 + theta5) - 0.5*a4*lc5_3*m5*theta_dot_2*sin(theta3 - 2.0*theta2 + theta4) - 0.5*a4*lc5_3*m5*theta_dot_2*sin(2.0*theta2 + theta3 + theta4) + 0.25*a4*lc5_3*m5*theta_dot_3*sin(theta3 - 2.0*theta2 + theta4) - 0.25*a4*lc5_3*m5*theta_dot_3*sin(2.0*theta2 + theta3 + theta4) - 0.5*a3*lc5_2*m5*theta_dot_3*sin(2.0*theta3 + theta4 + theta5) + 0.125*a3*lc5_2*m5*theta_dot_4*sin(theta4 - 2.0*theta2 + theta5) + 0.125*a3*lc5_2*m5*theta_dot_4*sin(2.0*theta2 + theta4 + theta5) + 0.25*a4*lc5_3*m5*theta_dot_4*sin(theta3 - 2.0*theta2 + theta4) - 0.25*a4*lc5_3*m5*theta_dot_4*sin(2.0*theta2 + theta3 + theta4) - 0.25*a3*lc5_2*m5*theta_dot_4*sin(2.0*theta3 + theta4 + theta5) + 0.125*a3*lc5_2*m5*theta_dot_5*sin(theta4 - 2.0*theta2 + theta5) + 0.125*a3*lc5_2*m5*theta_dot_5*sin(2.0*theta2 + theta4 + theta5) - 0.25*a3*lc5_2*m5*theta_dot_5*sin(2.0*theta3 + theta4 + theta5) - 0.125*a5*lc5_2*m5*theta_dot_2*cos(2.0*theta3 - 2*theta2 + 2.0*theta4 + 2.0*theta5) + 0.125*a5*lc5_2*m5*theta_dot_3*cos(2.0*theta3 - 2*theta2 + 2.0*theta4 + 2.0*theta5) + 0.125*a5*lc5_2*m5*theta_dot_4*cos(2.0*theta3 - 2*theta2 + 2.0*theta4 + 2.0*theta5) + 0.125*a5*lc5_2*m5*theta_dot_5*cos(2.0*theta3 - 2*theta2 + 2.0*theta4 + 2.0*theta5) - 0.25*a3*lc5_1*m5*theta_dot_2*cos(2.0*theta3 - 2.0*theta2 + theta4 + theta5) + 0.25*a3*lc5_1*m5*theta_dot_2*cos(2.0*theta2 + 2.0*theta3 + theta4 + theta5) + 0.25*a3*lc5_1*m5*theta_dot_3*cos(2.0*theta3 - 2.0*theta2 + theta4 + theta5) + 0.25*a3*lc5_1*m5*theta_dot_3*cos(2.0*theta2 + 2.0*theta3 + theta4 + theta5) + 0.125*a3*lc5_1*m5*theta_dot_4*cos(2.0*theta3 - 2.0*theta2 + theta4 + theta5) + 0.125*a3*lc5_1*m5*theta_dot_4*cos(2.0*theta2 + 2.0*theta3 + theta4 + theta5) + 0.125*a3*lc5_1*m5*theta_dot_5*cos(2.0*theta3 - 2.0*theta2 + theta4 + theta5) + 0.125*a3*lc5_1*m5*theta_dot_5*cos(2.0*theta2 + 2.0*theta3 + theta4 + theta5) + a1*lc2_1*m2*theta_dot_2*cos(theta2) - 0.5*a2*lc3_1*m3*theta_dot_3*cos(theta3) - 0.75*a3*lc4_2*m4*theta_dot_4*cos(theta4) + 0.75*a4*lc5_1*m5*theta_dot_5*cos(theta5) - 0.5*lc4_1*lc4_3*m4*theta_dot_2*sin(theta3 - 2.0*theta2 + theta4) - 0.5*lc4_1*lc4_3*m4*theta_dot_2*sin(2.0*theta2 + theta3 + theta4) + 0.25*lc4_1*lc4_3*m4*theta_dot_3*sin(theta3 - 2.0*theta2 + theta4) - 0.25*lc4_1*lc4_3*m4*theta_dot_3*sin(2.0*theta2 + theta3 + theta4) + 0.25*lc4_1*lc4_3*m4*theta_dot_4*sin(theta3 - 2.0*theta2 + theta4) - 0.25*lc4_1*lc4_3*m4*theta_dot_4*sin(2.0*theta2 + theta3 + theta4) - 0.375*a3*a4*m4*theta_dot_4*sin(theta4) - 0.75*a3*a4*m5*theta_dot_4*sin(theta4) - 0.25*lc5_1*lc5_2*m5*theta_dot_2*cos(2.0*theta3 - 2*theta2 + 2.0*theta4 + 2.0*theta5) + 0.25*lc5_1*lc5_2*m5*theta_dot_3*cos(2.0*theta3 - 2*theta2 + 2.0*theta4 + 2.0*theta5) + 0.25*lc5_1*lc5_2*m5*theta_dot_4*cos(2.0*theta3 - 2*theta2 + 2.0*theta4 + 2.0*theta5) + 0.25*lc5_1*lc5_2*m5*theta_dot_5*cos(2.0*theta3 - 2*theta2 + 2.0*theta4 + 2.0*theta5) - 0.25*a2*a3*m3*theta_dot_2*cos(2.0*theta2 - 1.0*theta3) + 0.125*a2*a3*m3*theta_dot_3*cos(2.0*theta2 - 1.0*theta3) - 0.5*a2*a3*m4*theta_dot_2*cos(2.0*theta2 - 1.0*theta3) + 0.25*a2*a3*m4*theta_dot_3*cos(2.0*theta2 - 1.0*theta3) - 0.5*a2*a3*m5*theta_dot_2*cos(2.0*theta2 - 1.0*theta3) + 0.25*a2*a3*m5*theta_dot_3*cos(2.0*theta2 - 1.0*theta3) + 0.125*a4*a5*m5*theta_dot_2*cos(2.0*theta2 - 1.0*theta5) - 0.0625*a4*a5*m5*theta_dot_5*cos(2.0*theta2 - 1.0*theta5) - 0.125*a5*lc5_1*m5*theta_dot_2*sin(2.0*theta3 - 2*theta2 + 2.0*theta4 + 2.0*theta5) + 0.125*a5*lc5_1*m5*theta_dot_3*sin(2.0*theta3 - 2*theta2 + 2.0*theta4 + 2.0*theta5) + 0.125*a5*lc5_1*m5*theta_dot_4*sin(2.0*theta3 - 2*theta2 + 2.0*theta4 + 2.0*theta5) + 0.125*a5*lc5_1*m5*theta_dot_5*sin(2.0*theta3 - 2*theta2 + 2.0*theta4 + 2.0*theta5) + 0.25*a3*lc5_2*m5*theta_dot_2*sin(2.0*theta3 - 2.0*theta2 + theta4 + theta5) - 0.25*a3*lc5_2*m5*theta_dot_2*sin(2.0*theta2 + 2.0*theta3 + theta4 + theta5) - 0.25*a3*lc5_2*m5*theta_dot_3*sin(2.0*theta3 - 2.0*theta2 + theta4 + theta5) - 0.25*a3*lc5_2*m5*theta_dot_3*sin(2.0*theta2 + 2.0*theta3 + theta4 + theta5) - 0.125*a3*lc5_2*m5*theta_dot_4*sin(2.0*theta3 - 2.0*theta2 + theta4 + theta5) - 0.125*a3*lc5_2*m5*theta_dot_4*sin(2.0*theta2 + 2.0*theta3 + theta4 + theta5) - 0.125*a3*lc5_2*m5*theta_dot_5*sin(2.0*theta3 - 2.0*theta2 + theta4 + theta5) - 0.125*a3*lc5_2*m5*theta_dot_5*sin(2.0*theta2 + 2.0*theta3 + theta4 + theta5) - 1.0*a1*lc2_3*m2*theta_dot_2*sin(theta2) - 1.0*a1*lc3_3*m3*theta_dot_2*sin(theta2) + 0.5*a2*lc3_2*m3*theta_dot_3*sin(theta3) - 1.0*a1*lc4_3*m4*theta_dot_2*sin(theta2) - 0.75*a3*lc4_1*m4*theta_dot_4*sin(theta4) - 1.0*a1*lc5_3*m5*theta_dot_2*sin(theta2) - 0.75*a4*lc5_2*m5*theta_dot_5*sin(theta5) + 0.25*a1*a5*m5*theta_dot_2*cos(theta3 - theta2 + theta4 + theta5) - 0.25*a1*a5*m5*theta_dot_3*cos(theta3 - theta2 + theta4 + theta5) - 0.25*a1*a5*m5*theta_dot_4*cos(theta3 - theta2 + theta4 + theta5) - 0.25*a1*a5*m5*theta_dot_5*cos(theta3 - theta2 + theta4 + theta5) - 0.5*a2*lc3_1*m3*theta_dot_2*cos(2.0*theta2 - 1.0*theta3) + 0.25*a2*lc3_1*m3*theta_dot_3*cos(2.0*theta2 - 1.0*theta3) - 0.25*a3*lc4_2*m4*theta_dot_2*cos(2.0*theta2 - 1.0*theta4) + 0.125*a3*lc4_2*m4*theta_dot_4*cos(2.0*theta2 - 1.0*theta4) + 0.25*a4*lc5_1*m5*theta_dot_2*cos(2.0*theta2 - 1.0*theta5) - 0.125*a4*lc5_1*m5*theta_dot_5*cos(2.0*theta2 - 1.0*theta5) + 0.125*a3*a4*m4*theta_dot_2*sin(2.0*theta2 - 1.0*theta4) + 0.25*a3*a4*m5*theta_dot_2*sin(2.0*theta2 - 1.0*theta4) - 0.0625*a3*a4*m4*theta_dot_4*sin(2.0*theta2 - 1.0*theta4) - 0.125*a3*a4*m5*theta_dot_4*sin(2.0*theta2 - 1.0*theta4)
C11 = C11a + C11b
C12a = - 1.0*I_xy_2*theta_dot_2*sin(theta2) - 0.25*I_xy_3*theta_dot_1*cos(2.0*theta2 - 2.0*theta3) + 0.25*I_xy_3*theta_dot_1*cos(2.0*theta2 + 2.0*theta3) - 0.5*I_yz_5*theta_dot_2*cos(theta3 - theta2 + theta4 + theta5) + 0.125*I_xx_3*theta_dot_1*sin(2.0*theta2 - 2.0*theta3) + 0.125*I_xx_3*theta_dot_1*sin(2.0*theta2 + 2.0*theta3) - 0.125*I_yy_3*theta_dot_1*sin(2.0*theta2 - 2.0*theta3) - 0.125*I_yy_3*theta_dot_1*sin(2.0*theta2 + 2.0*theta3) - 0.25*I_xy_4*theta_dot_1*cos(2.0*theta3 - 2.0*theta2 + 2.0*theta4) + 0.25*I_xy_4*theta_dot_1*cos(2.0*theta2 + 2.0*theta3 + 2.0*theta4) - 0.5*I_xz_5*theta_dot_2*sin(theta3 - theta2 + theta4 + theta5) - 0.5*I_xz_3*theta_dot_2*cos(theta2 - theta3) - 0.125*I_xx_4*theta_dot_1*sin(2.0*theta3 - 2.0*theta2 + 2.0*theta4) + 0.125*I_xx_4*theta_dot_1*sin(2.0*theta2 + 2.0*theta3 + 2.0*theta4) + 0.125*I_yy_4*theta_dot_1*sin(2.0*theta3 - 2.0*theta2 + 2.0*theta4) - 0.125*I_yy_4*theta_dot_1*sin(2.0*theta2 + 2.0*theta3 + 2.0*theta4) + 0.25*I_xy_5*theta_dot_1*cos(2.0*theta3 - 2.0*theta2 + 2.0*theta4 + 2.0*theta5) - 0.25*I_xy_5*theta_dot_1*cos(2.0*theta2 + 2.0*theta3 + 2.0*theta4 + 2.0*theta5) - 0.5*I_yz_3*theta_dot_2*sin(theta2 - theta3) - 0.5*I_xz_4*theta_dot_2*cos(theta2 + theta3 + theta4) + 0.125*I_xx_5*theta_dot_1*sin(2.0*theta3 - 2.0*theta2 + 2.0*theta4 + 2.0*theta5) - 0.125*I_xx_5*theta_dot_1*sin(2.0*theta2 + 2.0*theta3 + 2.0*theta4 + 2.0*theta5) - 0.125*I_yy_5*theta_dot_1*sin(2.0*theta3 - 2.0*theta2 + 2.0*theta4 + 2.0*theta5) + 0.125*I_yy_5*theta_dot_1*sin(2.0*theta2 + 2.0*theta3 + 2.0*theta4 + 2.0*theta5) + 0.5*I_yz_4*theta_dot_2*sin(theta2 + theta3 + theta4) - 0.5*I_xz_5*theta_dot_1*cos(theta3 - 2.0*theta2 + theta4 + theta5) - 0.5*I_xz_5*theta_dot_1*cos(2.0*theta2 + theta3 + theta4 + theta5) + 0.5*I_yz_5*theta_dot_1*sin(theta3 - 2.0*theta2 + theta4 + theta5) + 0.5*I_yz_5*theta_dot_1*sin(2.0*theta2 + theta3 + theta4 + theta5) + 0.25*I_xx_3*theta_dot_2*cos(theta2 - 2.0*theta3) - 0.25*I_xx_3*theta_dot_2*cos(theta2 + 2.0*theta3) - 0.25*I_xx_3*theta_dot_3*cos(theta2 - 2.0*theta3) - 0.25*I_xx_3*theta_dot_3*cos(theta2 + 2.0*theta3) - 0.25*I_yy_3*theta_dot_2*cos(theta2 - 2.0*theta3) + 0.25*I_yy_3*theta_dot_2*cos(theta2 + 2.0*theta3) + 0.5*I_yz_3*theta_dot_1*cos(2.0*theta2 + theta3) + 0.25*I_yy_3*theta_dot_3*cos(theta2 - 2.0*theta3) + 0.25*I_yy_3*theta_dot_3*cos(theta2 + 2.0*theta3) + 0.5*I_xy_3*theta_dot_2*sin(theta2 - 2.0*theta3) + 0.5*I_xy_3*theta_dot_2*sin(theta2 + 2.0*theta3) + 0.5*I_xz_3*theta_dot_1*sin(2.0*theta2 + theta3) - 0.5*I_xy_3*theta_dot_3*sin(theta2 - 2.0*theta3) + 0.5*I_xy_3*theta_dot_3*sin(theta2 + 2.0*theta3) - 0.25*I_xx_4*theta_dot_2*cos(theta2 + 2.0*theta3 + 2.0*theta4) - 0.25*I_xx_4*theta_dot_3*cos(theta2 + 2.0*theta3 + 2.0*theta4) - 0.25*I_xx_4*theta_dot_4*cos(theta2 + 2.0*theta3 + 2.0*theta4) + 0.25*I_yy_4*theta_dot_2*cos(theta2 + 2.0*theta3 + 2.0*theta4) + 0.25*I_yy_4*theta_dot_3*cos(theta2 + 2.0*theta3 + 2.0*theta4) + 0.25*I_yy_4*theta_dot_4*cos(theta2 + 2.0*theta3 + 2.0*theta4) + 0.5*I_xy_4*theta_dot_2*sin(theta2 + 2.0*theta3 + 2.0*theta4) + 0.5*I_xy_4*theta_dot_3*sin(theta2 + 2.0*theta3 + 2.0*theta4) + 0.5*I_xy_4*theta_dot_4*sin(theta2 + 2.0*theta3 + 2.0*theta4) + 0.25*I_xx_5*theta_dot_2*cos(theta2 + 2.0*theta3 + 2.0*theta4 + 2.0*theta5) + 0.25*I_xx_5*theta_dot_3*cos(theta2 + 2.0*theta3 + 2.0*theta4 + 2.0*theta5) + 0.25*I_xx_5*theta_dot_4*cos(theta2 + 2.0*theta3 + 2.0*theta4 + 2.0*theta5) + 0.25*I_xx_5*theta_dot_5*cos(theta2 + 2.0*theta3 + 2.0*theta4 + 2.0*theta5) - 0.25*I_yy_5*theta_dot_2*cos(theta2 + 2.0*theta3 + 2.0*theta4 + 2.0*theta5) - 0.25*I_yy_5*theta_dot_3*cos(theta2 + 2.0*theta3 + 2.0*theta4 + 2.0*theta5) - 0.25*I_yy_5*theta_dot_4*cos(theta2 + 2.0*theta3 + 2.0*theta4 + 2.0*theta5) - 0.25*I_yy_5*theta_dot_5*cos(theta2 + 2.0*theta3 + 2.0*theta4 + 2.0*theta5) - 1.0*I_xz_2*theta_dot_1*cos(2.0*theta2) - 0.5*I_xz_4*theta_dot_2*cos(theta3 - theta2 + theta4) - 0.5*I_xy_5*theta_dot_2*sin(theta2 + 2.0*theta3 + 2.0*theta4 + 2.0*theta5) - 0.5*I_xy_5*theta_dot_3*sin(theta2 + 2.0*theta3 + 2.0*theta4 + 2.0*theta5) - 0.5*I_xy_5*theta_dot_4*sin(theta2 + 2.0*theta3 + 2.0*theta4 + 2.0*theta5) - 0.5*I_xy_5*theta_dot_5*sin(theta2 + 2.0*theta3 + 2.0*theta4 + 2.0*theta5) - 0.5*I_xx_2*theta_dot_1*sin(2.0*theta2) - 0.25*I_xx_3*theta_dot_1*sin(2.0*theta2) - 0.25*I_xx_4*theta_dot_1*sin(2.0*theta2) - 0.25*I_xx_5*theta_dot_1*sin(2.0*theta2) - 0.25*I_yy_3*theta_dot_1*sin(2.0*theta2) - 0.25*I_yy_4*theta_dot_1*sin(2.0*theta2) - 0.25*I_yy_5*theta_dot_1*sin(2.0*theta2) + 0.5*I_zz_2*theta_dot_1*sin(2.0*theta2) + 0.5*I_zz_3*theta_dot_1*sin(2.0*theta2) + 0.5*I_zz_4*theta_dot_1*sin(2.0*theta2) + 0.5*I_zz_5*theta_dot_1*sin(2.0*theta2) + 0.5*I_yz_4*theta_dot_2*sin(theta3 - theta2 + theta4) - 0.5*I_yz_5*theta_dot_2*cos(theta2 + theta3 + theta4 + theta5) - 0.5*I_xz_5*theta_dot_2*sin(theta2 + theta3 + theta4 + theta5) + 0.5*I_yz_3*theta_dot_1*cos(2.0*theta2 - theta3) - 0.5*I_xz_3*theta_dot_2*cos(theta2 + theta3) - 0.5*I_xz_3*theta_dot_1*sin(2.0*theta2 - theta3) + 0.5*I_yz_3*theta_dot_2*sin(theta2 + theta3) + 0.25*I_xx_4*theta_dot_2*cos(2.0*theta3 - theta2 + 2.0*theta4) - 0.25*I_xx_4*theta_dot_3*cos(2.0*theta3 - theta2 + 2.0*theta4) - 0.25*I_xx_4*theta_dot_4*cos(2.0*theta3 - theta2 + 2.0*theta4) - 0.25*I_yy_4*theta_dot_2*cos(2.0*theta3 - theta2 + 2.0*theta4) + 0.25*I_yy_4*theta_dot_3*cos(2.0*theta3 - theta2 + 2.0*theta4) + 0.25*I_yy_4*theta_dot_4*cos(2.0*theta3 - theta2 + 2.0*theta4) + 0.5*I_yz_4*theta_dot_1*cos(theta3 - 2.0*theta2 + theta4) + 0.5*I_yz_4*theta_dot_1*cos(2.0*theta2 + theta3 + theta4) - 0.5*I_xy_4*theta_dot_2*sin(2.0*theta3 - theta2 + 2.0*theta4) + 0.5*I_xy_4*theta_dot_3*sin(2.0*theta3 - theta2 + 2.0*theta4) + 0.5*I_xy_4*theta_dot_4*sin(2.0*theta3 - theta2 + 2.0*theta4) + 0.5*I_xz_4*theta_dot_1*sin(theta3 - 2.0*theta2 + theta4) + 0.5*I_xz_4*theta_dot_1*sin(2.0*theta2 + theta3 + theta4) - 0.25*I_xx_5*theta_dot_2*cos(2.0*theta3 - theta2 + 2.0*theta4 + 2.0*theta5) + 0.25*I_xx_5*theta_dot_3*cos(2.0*theta3 - theta2 + 2.0*theta4 + 2.0*theta5) + 0.25*I_xx_5*theta_dot_4*cos(2.0*theta3 - theta2 + 2.0*theta4 + 2.0*theta5) + 0.25*I_xx_5*theta_dot_5*cos(2.0*theta3 - theta2 + 2.0*theta4 + 2.0*theta5) + 0.25*I_yy_5*theta_dot_2*cos(2.0*theta3 - theta2 + 2.0*theta4 + 2.0*theta5) - 0.25*I_yy_5*theta_dot_3*cos(2.0*theta3 - theta2 + 2.0*theta4 + 2.0*theta5) - 0.25*I_yy_5*theta_dot_4*cos(2.0*theta3 - theta2 + 2.0*theta4 + 2.0*theta5) - 0.25*I_yy_5*theta_dot_5*cos(2.0*theta3 - theta2 + 2.0*theta4 + 2.0*theta5) - 1.0*I_yz_2*theta_dot_2*cos(theta2) + 0.5*I_zz_3*theta_dot_3*cos(theta2) + 0.5*I_zz_4*theta_dot_3*cos(theta2) + 0.5*I_zz_4*theta_dot_4*cos(theta2) + 0.5*I_zz_5*theta_dot_3*cos(theta2) + 0.5*I_zz_5*theta_dot_4*cos(theta2) + 0.5*I_zz_5*theta_dot_5*cos(theta2) + 0.5*I_xy_5*theta_dot_2*sin(2.0*theta3 - theta2 + 2.0*theta4 + 2.0*theta5) - 0.5*I_xy_5*theta_dot_3*sin(2.0*theta3 - theta2 + 2.0*theta4 + 2.0*theta5) - 0.5*I_xy_5*theta_dot_4*sin(2.0*theta3 - theta2 + 2.0*theta4 + 2.0*theta5) - 0.5*I_xy_5*theta_dot_5*sin(2.0*theta3 - theta2 + 2.0*theta4 + 2.0*theta5) - 0.125*lc3_1^2*m3*theta_dot_1*sin(2.0*theta2 - 2.0*theta3) - 0.125*lc3_1^2*m3*theta_dot_1*sin(2.0*theta2 + 2.0*theta3) + 0.125*lc3_2^2*m3*theta_dot_1*sin(2.0*theta2 - 2.0*theta3) + 0.125*lc3_2^2*m3*theta_dot_1*sin(2.0*theta2 + 2.0*theta3) + 0.03125*a4^2*m4*theta_dot_1*sin(2.0*theta3 - 2.0*theta2 + 2.0*theta4) - 0.03125*a4^2*m4*theta_dot_1*sin(2.0*theta2 + 2.0*theta3 + 2.0*theta4) + 0.125*a4^2*m5*theta_dot_1*sin(2.0*theta3 - 2.0*theta2 + 2.0*theta4) - 0.125*a4^2*m5*theta_dot_1*sin(2.0*theta2 + 2.0*theta3 + 2.0*theta4) + 0.125*lc4_1^2*m4*theta_dot_1*sin(2.0*theta3 - 2.0*theta2 + 2.0*theta4) - 0.125*lc4_1^2*m4*theta_dot_1*sin(2.0*theta2 + 2.0*theta3 + 2.0*theta4) - 0.125*lc4_2^2*m4*theta_dot_1*sin(2.0*theta3 - 2.0*theta2 + 2.0*theta4) + 0.125*lc4_2^2*m4*theta_dot_1*sin(2.0*theta2 + 2.0*theta3 + 2.0*theta4) - 0.03125*a5^2*m5*theta_dot_1*sin(2.0*theta3 - 2.0*theta2 + 2.0*theta4 + 2.0*theta5) + 0.03125*a5^2*m5*theta_dot_1*sin(2.0*theta2 + 2.0*theta3 + 2.0*theta4 + 2.0*theta5) - 0.125*lc5_1^2*m5*theta_dot_1*sin(2.0*theta3 - 2.0*theta2 + 2.0*theta4 + 2.0*theta5) + 0.125*lc5_1^2*m5*theta_dot_1*sin(2.0*theta2 + 2.0*theta3 + 2.0*theta4 + 2.0*theta5) + 0.125*lc5_2^2*m5*theta_dot_1*sin(2.0*theta3 - 2.0*theta2 + 2.0*theta4 + 2.0*theta5) - 0.125*lc5_2^2*m5*theta_dot_1*sin(2.0*theta2 + 2.0*theta3 + 2.0*theta4 + 2.0*theta5) - 0.0625*a3^2*m3*theta_dot_2*cos(theta2 - 2.0*theta3) + 0.0625*a3^2*m3*theta_dot_2*cos(theta2 + 2.0*theta3) + 0.0625*a3^2*m3*theta_dot_3*cos(theta2 - 2.0*theta3) + 0.0625*a3^2*m3*theta_dot_3*cos(theta2 + 2.0*theta3) - 0.25*a3^2*m4*theta_dot_2*cos(theta2 - 2.0*theta3) + 0.25*a3^2*m4*theta_dot_2*cos(theta2 + 2.0*theta3) + 0.25*a3^2*m4*theta_dot_3*cos(theta2 - 2.0*theta3) + 0.25*a3^2*m4*theta_dot_3*cos(theta2 + 2.0*theta3) - 0.25*a3^2*m5*theta_dot_2*cos(theta2 - 2.0*theta3) + 0.25*a3^2*m5*theta_dot_2*cos(theta2 + 2.0*theta3) + 0.25*a3^2*m5*theta_dot_3*cos(theta2 - 2.0*theta3) + 0.25*a3^2*m5*theta_dot_3*cos(theta2 + 2.0*theta3) - 0.25*lc3_1^2*m3*theta_dot_2*cos(theta2 - 2.0*theta3) + 0.25*lc3_1^2*m3*theta_dot_2*cos(theta2 + 2.0*theta3) + 0.25*lc3_1^2*m3*theta_dot_3*cos(theta2 - 2.0*theta3) + 0.25*lc3_1^2*m3*theta_dot_3*cos(theta2 + 2.0*theta3) + 0.25*lc3_2^2*m3*theta_dot_2*cos(theta2 - 2.0*theta3) - 0.25*lc3_2^2*m3*theta_dot_2*cos(theta2 + 2.0*theta3) - 0.25*lc3_2^2*m3*theta_dot_3*cos(theta2 - 2.0*theta3) - 0.25*lc3_2^2*m3*theta_dot_3*cos(theta2 + 2.0*theta3) + 0.0625*a4^2*m4*theta_dot_2*cos(theta2 + 2.0*theta3 + 2.0*theta4) + 0.0625*a4^2*m4*theta_dot_3*cos(theta2 + 2.0*theta3 + 2.0*theta4) + 0.25*a4^2*m5*theta_dot_2*cos(theta2 + 2.0*theta3 + 2.0*theta4) + 0.0625*a4^2*m4*theta_dot_4*cos(theta2 + 2.0*theta3 + 2.0*theta4) + 0.25*a4^2*m5*theta_dot_3*cos(theta2 + 2.0*theta3 + 2.0*theta4) + 0.25*a4^2*m5*theta_dot_4*cos(theta2 + 2.0*theta3 + 2.0*theta4) + 0.25*lc4_1^2*m4*theta_dot_2*cos(theta2 + 2.0*theta3 + 2.0*theta4) + 0.25*lc4_1^2*m4*theta_dot_3*cos(theta2 + 2.0*theta3 + 2.0*theta4) - 0.25*lc4_2^2*m4*theta_dot_2*cos(theta2 + 2.0*theta3 + 2.0*theta4) + 0.25*lc4_1^2*m4*theta_dot_4*cos(theta2 + 2.0*theta3 + 2.0*theta4) - 0.25*lc4_2^2*m4*theta_dot_3*cos(theta2 + 2.0*theta3 + 2.0*theta4) - 0.25*lc4_2^2*m4*theta_dot_4*cos(theta2 + 2.0*theta3 + 2.0*theta4) - 0.0625*a5^2*m5*theta_dot_2*cos(theta2 + 2.0*theta3 + 2.0*theta4 + 2.0*theta5) - 0.0625*a5^2*m5*theta_dot_3*cos(theta2 + 2.0*theta3 + 2.0*theta4 + 2.0*theta5) - 0.0625*a5^2*m5*theta_dot_4*cos(theta2 + 2.0*theta3 + 2.0*theta4 + 2.0*theta5) - 0.0625*a5^2*m5*theta_dot_5*cos(theta2 + 2.0*theta3 + 2.0*theta4 + 2.0*theta5) - 0.25*lc5_1^2*m5*theta_dot_2*cos(theta2 + 2.0*theta3 + 2.0*theta4 + 2.0*theta5) - 0.25*lc5_1^2*m5*theta_dot_3*cos(theta2 + 2.0*theta3 + 2.0*theta4 + 2.0*theta5) + 0.25*lc5_2^2*m5*theta_dot_2*cos(theta2 + 2.0*theta3 + 2.0*theta4 + 2.0*theta5) - 0.25*lc5_1^2*m5*theta_dot_4*cos(theta2 + 2.0*theta3 + 2.0*theta4 + 2.0*theta5) + 0.25*lc5_2^2*m5*theta_dot_3*cos(theta2 + 2.0*theta3 + 2.0*theta4 + 2.0*theta5) - 0.25*lc5_1^2*m5*theta_dot_5*cos(theta2 + 2.0*theta3 + 2.0*theta4 + 2.0*theta5) + 0.25*lc5_2^2*m5*theta_dot_4*cos(theta2 + 2.0*theta3 + 2.0*theta4 + 2.0*theta5) + 0.25*lc5_2^2*m5*theta_dot_5*cos(theta2 + 2.0*theta3 + 2.0*theta4 + 2.0*theta5) + 0.125*a2^2*m2*theta_dot_1*sin(2.0*theta2) + 0.5*a2^2*m3*theta_dot_1*sin(2.0*theta2) + 0.5*a2^2*m4*theta_dot_1*sin(2.0*theta2) + 0.0625*a3^2*m3*theta_dot_1*sin(2.0*theta2) + 0.5*a2^2*m5*theta_dot_1*sin(2.0*theta2) + 0.25*a3^2*m4*theta_dot_1*sin(2.0*theta2) + 0.25*a3^2*m5*theta_dot_1*sin(2.0*theta2) + 0.0625*a4^2*m4*theta_dot_1*sin(2.0*theta2) + 0.25*a4^2*m5*theta_dot_1*sin(2.0*theta2) + 0.0625*a5^2*m5*theta_dot_1*sin(2.0*theta2) + 0.5*lc2_1^2*m2*theta_dot_1*sin(2.0*theta2) - 0.5*lc2_3^2*m2*theta_dot_1*sin(2.0*theta2) + 0.25*lc3_1^2*m3*theta_dot_1*sin(2.0*theta2) + 0.25*lc3_2^2*m3*theta_dot_1*sin(2.0*theta2) - 0.5*lc3_3^2*m3*theta_dot_1*sin(2.0*theta2) + 0.25*lc4_1^2*m4*theta_dot_1*sin(2.0*theta2) + 0.25*lc4_2^2*m4*theta_dot_1*sin(2.0*theta2) - 0.5*lc4_3^2*m4*theta_dot_1*sin(2.0*theta2) + 0.25*lc5_1^2*m5*theta_dot_1*sin(2.0*theta2) + 0.25*lc5_2^2*m5*theta_dot_1*sin(2.0*theta2) - 0.5*lc5_3^2*m5*theta_dot_1*sin(2.0*theta2) - 0.0625*a4^2*m4*theta_dot_2*cos(2.0*theta3 - theta2 + 2.0*theta4) + 0.0625*a4^2*m4*theta_dot_3*cos(2.0*theta3 - theta2 + 2.0*theta4) - 0.25*a4^2*m5*theta_dot_2*cos(2.0*theta3 - theta2 + 2.0*theta4) + 0.0625*a4^2*m4*theta_dot_4*cos(2.0*theta3 - theta2 + 2.0*theta4) + 0.25*a4^2*m5*theta_dot_3*cos(2.0*theta3 - theta2 + 2.0*theta4) + 0.25*a4^2*m5*theta_dot_4*cos(2.0*theta3 - theta2 + 2.0*theta4) - 0.25*lc4_1^2*m4*theta_dot_2*cos(2.0*theta3 - theta2 + 2.0*theta4) + 0.25*lc4_1^2*m4*theta_dot_3*cos(2.0*theta3 - theta2 + 2.0*theta4) + 0.25*lc4_2^2*m4*theta_dot_2*cos(2.0*theta3 - theta2 + 2.0*theta4) + 0.25*lc4_1^2*m4*theta_dot_4*cos(2.0*theta3 - theta2 + 2.0*theta4) - 0.25*lc4_2^2*m4*theta_dot_3*cos(2.0*theta3 - theta2 + 2.0*theta4) - 0.25*lc4_2^2*m4*theta_dot_4*cos(2.0*theta3 - theta2 + 2.0*theta4) + 0.0625*a5^2*m5*theta_dot_2*cos(2.0*theta3 - theta2 + 2.0*theta4 + 2.0*theta5) - 0.0625*a5^2*m5*theta_dot_3*cos(2.0*theta3 - theta2 + 2.0*theta4 + 2.0*theta5) - 0.0625*a5^2*m5*theta_dot_4*cos(2.0*theta3 - theta2 + 2.0*theta4 + 2.0*theta5) - 0.0625*a5^2*m5*theta_dot_5*cos(2.0*theta3 - theta2 + 2.0*theta4 + 2.0*theta5) + 0.125*a3^2*m3*theta_dot_3*cos(theta2) + 0.5*a3^2*m4*theta_dot_3*cos(theta2) + 0.5*a3^2*m5*theta_dot_3*cos(theta2) + 0.125*a4^2*m4*theta_dot_3*cos(theta2) + 0.125*a4^2*m4*theta_dot_4*cos(theta2) + 0.5*a4^2*m5*theta_dot_3*cos(theta2) + 0.5*a4^2*m5*theta_dot_4*cos(theta2) + 0.125*a5^2*m5*theta_dot_3*cos(theta2) + 0.125*a5^2*m5*theta_dot_4*cos(theta2) + 0.125*a5^2*m5*theta_dot_5*cos(theta2) + 0.25*lc5_1^2*m5*theta_dot_2*cos(2.0*theta3 - theta2 + 2.0*theta4 + 2.0*theta5) - 0.25*lc5_1^2*m5*theta_dot_3*cos(2.0*theta3 - theta2 + 2.0*theta4 + 2.0*theta5) - 0.25*lc5_2^2*m5*theta_dot_2*cos(2.0*theta3 - theta2 + 2.0*theta4 + 2.0*theta5) - 0.25*lc5_1^2*m5*theta_dot_4*cos(2.0*theta3 - theta2 + 2.0*theta4 + 2.0*theta5) + 0.25*lc5_2^2*m5*theta_dot_3*cos(2.0*theta3 - theta2 + 2.0*theta4 + 2.0*theta5) - 0.25*lc5_1^2*m5*theta_dot_5*cos(2.0*theta3 - theta2 + 2.0*theta4 + 2.0*theta5) + 0.25*lc5_2^2*m5*theta_dot_4*cos(2.0*theta3 - theta2 + 2.0*theta4 + 2.0*theta5) + 0.25*lc5_2^2*m5*theta_dot_5*cos(2.0*theta3 - theta2 + 2.0*theta4 + 2.0*theta5) + 0.5*lc3_1^2*m3*theta_dot_3*cos(theta2) + 0.5*lc3_2^2*m3*theta_dot_3*cos(theta2) + 0.5*lc4_1^2*m4*theta_dot_3*cos(theta2) + 0.5*lc4_1^2*m4*theta_dot_4*cos(theta2) + 0.5*lc4_2^2*m4*theta_dot_3*cos(theta2) + 0.5*lc4_2^2*m4*theta_dot_4*cos(theta2) + 0.5*lc5_1^2*m5*theta_dot_3*cos(theta2) + 0.5*lc5_1^2*m5*theta_dot_4*cos(theta2) + 0.5*lc5_2^2*m5*theta_dot_3*cos(theta2) + 0.5*lc5_1^2*m5*theta_dot_5*cos(theta2) + 0.5*lc5_2^2*m5*theta_dot_4*cos(theta2) + 0.5*lc5_2^2*m5*theta_dot_5*cos(theta2) - 0.03125*a3^2*m3*theta_dot_1*sin(2.0*theta2 - 2.0*theta3) - 0.03125*a3^2*m3*theta_dot_1*sin(2.0*theta2 + 2.0*theta3) - 0.125*a3^2*m4*theta_dot_1*sin(2.0*theta2 - 2.0*theta3) - 0.125*a3^2*m4*theta_dot_1*sin(2.0*theta2 + 2.0*theta3) - 0.125*a3^2*m5*theta_dot_1*sin(2.0*theta2 - 2.0*theta3) - 0.125*a3^2*m5*theta_dot_1*sin(2.0*theta2 + 2.0*theta3) + 1.0*lc2_1*lc2_2*m2*theta_dot_2*sin(theta2) + 0.5*a1*lc5_1*m5*theta_dot_1*cos(theta3 - theta2 + theta4 + theta5) + 0.5*a2*lc5_1*m5*theta_dot_2*cos(theta3 - theta2 + theta4 + theta5) + 0.25*lc3_1*lc3_2*m3*theta_dot_1*cos(2.0*theta2 - 2.0*theta3) - 0.25*lc3_1*lc3_2*m3*theta_dot_1*cos(2.0*theta2 + 2.0*theta3) - 0.125*a3*lc3_1*m3*theta_dot_1*sin(2.0*theta2 - 2.0*theta3) - 0.125*a3*lc3_1*m3*theta_dot_1*sin(2.0*theta2 + 2.0*theta3) + 0.125*a4*lc4_2*m4*theta_dot_1*cos(2.0*theta3 - 2.0*theta2 + 2.0*theta4) - 0.125*a4*lc4_2*m4*theta_dot_1*cos(2.0*theta2 + 2.0*theta3 + 2.0*theta4) + 0.5*lc5_2*lc5_3*m5*theta_dot_2*cos(theta3 - theta2 + theta4 + theta5) + 0.25*a3*a4*m4*theta_dot_3*cos(theta2 - theta4) + 0.125*a3*a4*m4*theta_dot_4*cos(theta2 - theta4) + 0.5*a3*a4*m5*theta_dot_3*cos(theta2 - theta4) + 0.25*a3*a4*m5*theta_dot_4*cos(theta2 - theta4) - 0.5*a1*lc5_2*m5*theta_dot_1*sin(theta3 - theta2 + theta4 + theta5) - 0.5*a2*lc5_2*m5*theta_dot_2*sin(theta3 - theta2 + theta4 + theta5) + 0.25*a5*lc5_3*m5*theta_dot_2*sin(theta3 - theta2 + theta4 + theta5) + 0.25*lc4_1*lc4_2*m4*theta_dot_1*cos(2.0*theta3 - 2.0*theta2 + 2.0*theta4) - 0.25*lc4_1*lc4_2*m4*theta_dot_1*cos(2.0*theta2 + 2.0*theta3 + 2.0*theta4) - 0.5*a1*lc3_2*m3*theta_dot_1*cos(theta2 - theta3) - 0.5*a2*lc3_2*m3*theta_dot_2*cos(theta2 - theta3) + 0.25*a3*lc3_3*m3*theta_dot_2*cos(theta2 - theta3) + 0.5*a3*lc4_1*m4*theta_dot_3*cos(theta2 - theta4) + 0.5*a3*lc4_3*m4*theta_dot_2*cos(theta2 - theta3) + 0.25*a3*lc4_1*m4*theta_dot_4*cos(theta2 - theta4) + 0.5*a3*lc5_3*m5*theta_dot_2*cos(theta2 - theta3) + 0.5*a4*lc5_2*m5*theta_dot_3*cos(theta2 - theta5) + 0.5*a4*lc5_2*m5*theta_dot_4*cos(theta2 - theta5) + 0.25*a4*lc5_2*m5*theta_dot_5*cos(theta2 - theta5) 
